simulink model "Australian14gen_original"  (R2017a)
settings: Solver=ode23tb  StartTime=0.0  StopTime=70  MaxStep=1/60  RelTol=1e-3  AbsTol=1e-1  EnableMultiTasking=on
PreLoadFcn:
  | dataaustralian14gen
values from neighbouring files (symbols this model uses):
  bus_v = [ 101	15 ... (first row only)    [dataaustralian14gen.m]
  comp = [ 1	211	0	0 ... (first row only)    [dataaustralian14gen.m]
  Exc = [ 101	0	 200	0.1	    13.25  2.5	 0	0       0       0       0       0 ... (first row only)    [dataaustralian14gen.m]
  FH = 13    [dataaustralian14gen.m]
  FI = 1    [dataaustralian14gen.m]
  FL = .1    (= 0.1)    [dataaustralian14gen.m]
  G_data = [ 101	333.3	15	3.6	0.14	1.1	0.65	0.25	8.5     0.25	0.05	0       0       0.25	0.2 	0 ... (first row only)    [dataaustralian14gen.m]
  KH = 120    [dataaustralian14gen.m]
  KI = 10    [dataaustralian14gen.m]
  KL = 10    [dataaustralian14gen.m]
  line = [ 102	217	0.0084	0.0667	0.817	330	1 ... (first row only)    [dataaustralian14gen.m]
  p = p_case4    [dataaustralian14gen.m]
  PSSMODEL = 1    [dataaustralian14gen.m]
  trans = [ 1	101	102	15	330	333.3	12	12 ... (first row only)    [dataaustralian14gen.m]
undefined symbols (not defined in the file or in its folder): D1, Delta
libraries: powerlib x297, sps_avr x14, factslib x5, powerlib_extras x4
(part 1 of 3)
Description:
  | SimPowerSystem model of the Simplified 14-Generator model
  | of the SE Australian Power System developed by Mike Gibbard & David Vowles,
  | School of Electrical & Electronic Engineering, The university of Adelaide, south australia)
  | 
  | SimPowerSystems model and validations by Ali Moeini and Innocent Kamwa,
  | IREQ, Hydro-Québec, Canada
settings Model: Creator=IREQ  LastModifiedBy=dominic
settings DataIOCC: LimitDataPoints=on  SaveFormat=Array
settings OptimizationCC: ExpressionDepthLimit=2147483647  LifeSpan=inf
settings DebuggingCC: UnderspecifiedInitializationDetection=Classic  MergeDetectMultiDrivingBlocksExec=none  IgnoredZcDiagnostic=none  SolverPrmCheckMsg=warning  UnconnectedInputMsg=none  UnconnectedOutputMsg=none  UnconnectedLineMsg=none  StateNameClashWarn=warning  SFUnexpectedBacktrackingDiag=warning  SFNoUnconditionalDefaultTransitionDiag=warning  SFExecutionAtInitializationDiag=none
settings HardwareCC: ProdBitPerPointer=32  ProdBitPerSizeT=32  ProdBitPerPtrDiffT=32  ProdLargestAtomicFloat=None  ProdIntDivRoundTo=Undefined  ProdEndianess=Unspecified  ProdWordSize=32  ProdHWDeviceType=32-bit Generic
settings ModelReferenceCC: PropagateSignalLabelsOutOfModel=off
settings GRTTargetCC: TargetLangStandard=C89/C90 (ANSI)  GeneratePreprocessorConditionals=Disable all
settings ConfigComp: CovMetricSettings=dw  CovHtmlReporting=on  CovSaveCumulativeToWorkspaceVar=on  CovSaveSingleToWorkspaceVar=on  CovExternalEMLEnable=off  CovSFcnEnable=off

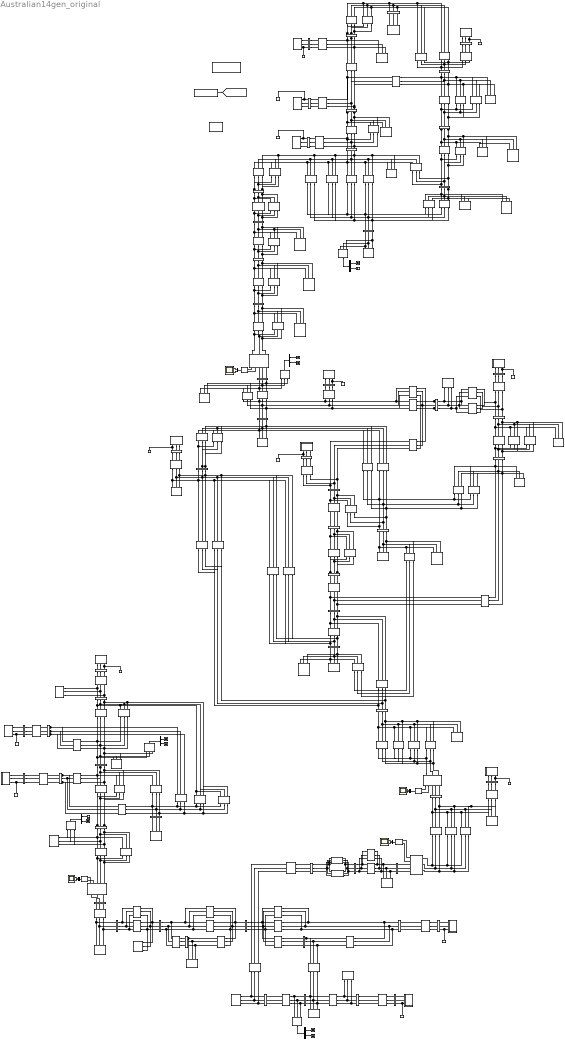
== system Australian14gen_original ==
  1 : powerlib/Elements/Three-Phase Series RLC Branch  LConnTagsString=A|B|C  RConnTagsString=A|B|C  BranchType=C  Resistance=0  Inductance=0  Capacitance=1/(0.0337)/(2*pi*50)*(330^2/100)  Measurements=None
  2 : powerlib/Elements/Three-Phase Series RLC Branch  LConnTagsString=A|B|C  RConnTagsString=A|B|C  BranchType=C  Resistance=0  Inductance=0  Capacitance=1/(0.0337)/(2*pi*50)*(330^2/100)  Measurements=None
  3-Phase Active & Reactive Power (Phasor Type){1..4} (4 alike) : powerlib_extras/Phasor Library/3-Phase Active & Reactive Power (Phasor Type)
      settings: SourceProductName=The database /home/dominic/.matlab/R2017a/slblocks_master.db is locked, or a table in the database is locked. (database is locked)
  B101 : powerlib/Measurements/Three-Phase V-I Measurement  VoltageMeasurement=phase-to-phase  SetLabelV=on  LabelV=Vabc_B101  Vpu=off  VpuLL=off  CurrentMeasurement=no  SetLabelI=on  LabelI=Iabc_B101  Ipu=off  Pbase=100e6  Vbase=bus_v(1,2)*e3  OutputType=Complex  PhasorSimulation=on  PSBequivalent=0
  B102 : powerlib/Measurements/Three-Phase V-I Measurement  VoltageMeasurement=phase-to-ground  SetLabelV=on  LabelV=Vabc_B102  Vpu=off  VpuLL=off  CurrentMeasurement=yes  SetLabelI=on  LabelI=Iabc_B102  Ipu=off  Pbase=100e6  Vbase=bus_v(2,2)*e3  OutputType=Complex  PhasorSimulation=on  PSBequivalent=0
  B201 : powerlib/Measurements/Three-Phase V-I Measurement  VoltageMeasurement=phase-to-phase  SetLabelV=on  LabelV=Vabc_B201  Vpu=off  VpuLL=off  CurrentMeasurement=no  SetLabelI=on  LabelI=Iabc_B201  Ipu=off  Pbase=100e6  Vbase=bus_v(3,2)*e3  OutputType=Complex  PhasorSimulation=on  PSBequivalent=0
  B202 : powerlib/Measurements/Three-Phase V-I Measurement  VoltageMeasurement=phase-to-phase  SetLabelV=on  LabelV=Vabc_B202  Vpu=off  VpuLL=off  CurrentMeasurement=no  SetLabelI=on  LabelI=Iabc_B202  Ipu=off  Pbase=100e6  Vbase=bus_v(4,2)*e3  OutputType=Complex  PhasorSimulation=on  PSBequivalent=0
  B203 : powerlib/Measurements/Three-Phase V-I Measurement  VoltageMeasurement=phase-to-phase  SetLabelV=on  LabelV=Vabc_B203  Vpu=off  VpuLL=off  CurrentMeasurement=no  SetLabelI=on  LabelI=Iabc_B203  Ipu=off  Pbase=100e6  Vbase=bus_v(5,2)*e3  OutputType=Complex  PhasorSimulation=on  PSBequivalent=0
  B204 : powerlib/Measurements/Three-Phase V-I Measurement  VoltageMeasurement=phase-to-phase  SetLabelV=on  LabelV=Vabc_B204  Vpu=off  VpuLL=off  CurrentMeasurement=no  SetLabelI=on  LabelI=Iabc_B204  Ipu=off  Pbase=100e6  Vbase=bus_v(6,2)*e3  OutputType=Complex  PhasorSimulation=on  PSBequivalent=0
  B205 : powerlib/Measurements/Three-Phase V-I Measurement  VoltageMeasurement=phase-to-ground  SetLabelV=on  LabelV=Vabc_B205  Vpu=off  VpuLL=off  CurrentMeasurement=yes  SetLabelI=on  LabelI=Iabc_B205  Ipu=off  Pbase=100e6  Vbase=bus_v(7,2)*e3  OutputType=Complex  PhasorSimulation=on  PSBequivalent=0
  B206 : powerlib/Measurements/Three-Phase V-I Measurement  VoltageMeasurement=phase-to-ground  SetLabelV=on  LabelV=Vabc_B206  Vpu=off  VpuLL=off  CurrentMeasurement=yes  SetLabelI=on  LabelI=Iabc_B206  Ipu=off  Pbase=100e6  Vbase=bus_v(8,2)*e3  OutputType=Complex  PhasorSimulation=on  PSBequivalent=0
  B207 : powerlib/Measurements/Three-Phase V-I Measurement  VoltageMeasurement=phase-to-ground  SetLabelV=on  LabelV=Vabc_B207  Vpu=off  VpuLL=off  CurrentMeasurement=yes  SetLabelI=on  LabelI=Iabc_B207  Ipu=off  Pbase=100e6  Vbase=138e3  OutputType=Complex  PhasorSimulation=on  PSBequivalent=0
  B208 : powerlib/Measurements/Three-Phase V-I Measurement  VoltageMeasurement=phase-to-ground  SetLabelV=on  LabelV=Vabc_B208  Vpu=off  VpuLL=off  CurrentMeasurement=yes  SetLabelI=on  LabelI=Iabc_B208  Ipu=off  Pbase=100e6  Vbase=138e3  OutputType=Complex  PhasorSimulation=on  PSBequivalent=0
  B209 : powerlib/Measurements/Three-Phase V-I Measurement  VoltageMeasurement=phase-to-ground  SetLabelV=on  LabelV=Vabc_B209  Vpu=off  VpuLL=off  CurrentMeasurement=yes  SetLabelI=on  LabelI=Iabc_B209  Ipu=off  Pbase=100e6  Vbase=138e3  OutputType=Complex  PhasorSimulation=on  PSBequivalent=0
  B210 : powerlib/Measurements/Three-Phase V-I Measurement  VoltageMeasurement=phase-to-ground  SetLabelV=on  LabelV=Vabc_B210  Vpu=off  VpuLL=off  CurrentMeasurement=yes  SetLabelI=on  LabelI=Iabc_B210  Ipu=off  Pbase=100e6  Vbase=138e3  OutputType=Complex  PhasorSimulation=on  PSBequivalent=0
  B211 : powerlib/Measurements/Three-Phase V-I Measurement  VoltageMeasurement=phase-to-ground  SetLabelV=on  LabelV=Vabc_B211  Vpu=off  VpuLL=off  CurrentMeasurement=yes  SetLabelI=on  LabelI=Iabc_B211  Ipu=off  Pbase=100e6  Vbase=138e3  OutputType=Complex  PhasorSimulation=on  PSBequivalent=0
  B212 : powerlib/Measurements/Three-Phase V-I Measurement  VoltageMeasurement=phase-to-ground  SetLabelV=on  LabelV=Vabc_B212  Vpu=off  VpuLL=off  CurrentMeasurement=yes  SetLabelI=on  LabelI=Iabc_B212  Ipu=off  Pbase=100e6  Vbase=138e3  OutputType=Complex  PhasorSimulation=on  PSBequivalent=0
  B213 : powerlib/Measurements/Three-Phase V-I Measurement  VoltageMeasurement=phase-to-ground  SetLabelV=on  LabelV=Vabc_B213  Vpu=off  VpuLL=off  CurrentMeasurement=yes  SetLabelI=on  LabelI=Iabc_B213  Ipu=off  Pbase=100e6  Vbase=138e3  OutputType=Complex  PhasorSimulation=on  PSBequivalent=0
  B214 : powerlib/Measurements/Three-Phase V-I Measurement  VoltageMeasurement=phase-to-ground  SetLabelV=on  LabelV=Vabc_B214  Vpu=off  VpuLL=off  CurrentMeasurement=yes  SetLabelI=on  LabelI=Iabc_B214  Ipu=off  Pbase=100e6  Vbase=138e3  OutputType=Complex  PhasorSimulation=on  PSBequivalent=0
  B215 : powerlib/Measurements/Three-Phase V-I Measurement  VoltageMeasurement=phase-to-ground  SetLabelV=on  LabelV=Vabc_B215  Vpu=off  VpuLL=off  CurrentMeasurement=yes  SetLabelI=on  LabelI=Iabc_B215  Ipu=off  Pbase=100e6  Vbase=138e3  OutputType=Complex  PhasorSimulation=on  PSBequivalent=0
  B216 : powerlib/Measurements/Three-Phase V-I Measurement  VoltageMeasurement=phase-to-ground  SetLabelV=on  LabelV=Vabc_B216  Vpu=off  VpuLL=off  CurrentMeasurement=yes  SetLabelI=on  LabelI=Iabc_B216  Ipu=off  Pbase=100e6  Vbase=138e3  OutputType=Complex  PhasorSimulation=on  PSBequivalent=0
  B217 : powerlib/Measurements/Three-Phase V-I Measurement  VoltageMeasurement=phase-to-ground  SetLabelV=on  LabelV=Vabc_B217  Vpu=off  VpuLL=off  CurrentMeasurement=yes  SetLabelI=on  LabelI=Iabc_B217  Ipu=off  Pbase=100e6  Vbase=138e3  OutputType=Complex  PhasorSimulation=on  PSBequivalent=0
  B301 : powerlib/Measurements/Three-Phase V-I Measurement  VoltageMeasurement=phase-to-phase  SetLabelV=on  LabelV=Vabc_B301  Vpu=off  VpuLL=off  CurrentMeasurement=no  SetLabelI=on  LabelI=Iabc_B301  Ipu=off  Pbase=100e6  Vbase=138e3  OutputType=Complex  PhasorSimulation=on  PSBequivalent=0
  B302 : powerlib/Measurements/Three-Phase V-I Measurement  VoltageMeasurement=phase-to-phase  SetLabelV=on  LabelV=Vabc_B302  Vpu=off  VpuLL=off  CurrentMeasurement=no  SetLabelI=on  LabelI=Iabc_B302  Ipu=off  Pbase=100e6  Vbase=138e3  OutputType=Complex  PhasorSimulation=on  PSBequivalent=0
  B303 : powerlib/Measurements/Three-Phase V-I Measurement  VoltageMeasurement=phase-to-ground  SetLabelV=on  LabelV=Vabc_B303  Vpu=off  VpuLL=off  CurrentMeasurement=yes  SetLabelI=on  LabelI=Iabc_B303  Ipu=off  Pbase=100e6  Vbase=138e3  OutputType=Complex  PhasorSimulation=on  PSBequivalent=0
  B304 : powerlib/Measurements/Three-Phase V-I Measurement  VoltageMeasurement=phase-to-ground  SetLabelV=on  LabelV=Vabc_B304  Vpu=off  VpuLL=off  CurrentMeasurement=yes  SetLabelI=on  LabelI=Iabc_B304  Ipu=off  Pbase=100e6  Vbase=138e3  OutputType=Complex  PhasorSimulation=on  PSBequivalent=0
  B305 : powerlib/Measurements/Three-Phase V-I Measurement  VoltageMeasurement=phase-to-ground  SetLabelV=on  LabelV=Vabc_B305  Vpu=off  VpuLL=off  CurrentMeasurement=yes  SetLabelI=on  LabelI=Iabc_B305  Ipu=off  Pbase=100e6  Vbase=138e3  OutputType=Complex  PhasorSimulation=on  PSBequivalent=0
  B306 : powerlib/Measurements/Three-Phase V-I Measurement  VoltageMeasurement=phase-to-ground  SetLabelV=on  LabelV=Vabc_B306  Vpu=off  VpuLL=off  CurrentMeasurement=yes  SetLabelI=on  LabelI=Iabc_B306  Ipu=off  Pbase=100e6  Vbase=138e3  OutputType=Complex  PhasorSimulation=on  PSBequivalent=0
  B307 : powerlib/Measurements/Three-Phase V-I Measurement  VoltageMeasurement=phase-to-ground  SetLabelV=on  LabelV=Vabc_B307  Vpu=off  VpuLL=off  CurrentMeasurement=yes  SetLabelI=on  LabelI=Iabc_B307  Ipu=off  Pbase=100e6  Vbase=138e3  OutputType=Complex  PhasorSimulation=on  PSBequivalent=0
  B308 : powerlib/Measurements/Three-Phase V-I Measurement  VoltageMeasurement=phase-to-ground  SetLabelV=on  LabelV=Vabc_B308  Vpu=off  VpuLL=off  CurrentMeasurement=yes  SetLabelI=on  LabelI=Iabc_B308  Ipu=off  Pbase=100e6  Vbase=138e3  OutputType=Complex  PhasorSimulation=on  PSBequivalent=0
  B309 : powerlib/Measurements/Three-Phase V-I Measurement  VoltageMeasurement=phase-to-ground  SetLabelV=on  LabelV=Vabc_B309  Vpu=off  VpuLL=off  CurrentMeasurement=yes  SetLabelI=on  LabelI=Iabc_B309  Ipu=off  Pbase=100e6  Vbase=138e3  OutputType=Complex  PhasorSimulation=on  PSBequivalent=0
  B310 : powerlib/Measurements/Three-Phase V-I Measurement  VoltageMeasurement=phase-to-ground  SetLabelV=on  LabelV=Vabc_B310  Vpu=off  VpuLL=off  CurrentMeasurement=yes  SetLabelI=on  LabelI=Iabc_B310  Ipu=off  Pbase=100e6  Vbase=138e3  OutputType=Complex  PhasorSimulation=on  PSBequivalent=0
  B311 : powerlib/Measurements/Three-Phase V-I Measurement  VoltageMeasurement=phase-to-ground  SetLabelV=on  LabelV=Vabc_B311  Vpu=off  VpuLL=off  CurrentMeasurement=yes  SetLabelI=on  LabelI=Iabc_B311  Ipu=off  Pbase=100e6  Vbase=138e3  OutputType=Complex  PhasorSimulation=on  PSBequivalent=0
  B312 : powerlib/Measurements/Three-Phase V-I Measurement  VoltageMeasurement=phase-to-ground  SetLabelV=on  LabelV=Vabc_B312  Vpu=off  VpuLL=off  CurrentMeasurement=yes  SetLabelI=on  LabelI=Iabc_B312  Ipu=off  Pbase=100e6  Vbase=138e3  OutputType=Complex  PhasorSimulation=on  PSBequivalent=0
  B313 : powerlib/Measurements/Three-Phase V-I Measurement  VoltageMeasurement=phase-to-ground  SetLabelV=on  LabelV=Vabc_B313  Vpu=off  VpuLL=off  CurrentMeasurement=yes  SetLabelI=on  LabelI=Iabc_B313  Ipu=off  Pbase=100e6  Vbase=138e3  OutputType=Complex  PhasorSimulation=on  PSBequivalent=0
  B314 : powerlib/Measurements/Three-Phase V-I Measurement  VoltageMeasurement=phase-to-ground  SetLabelV=on  LabelV=Vabc_B314  Vpu=off  VpuLL=off  CurrentMeasurement=yes  SetLabelI=on  LabelI=Iabc_B314  Ipu=off  Pbase=100e6  Vbase=138e3  OutputType=Complex  PhasorSimulation=on  PSBequivalent=0
  B315 : powerlib/Measurements/Three-Phase V-I Measurement  VoltageMeasurement=phase-to-ground  SetLabelV=on  LabelV=Vabc_B315  Vpu=off  VpuLL=off  CurrentMeasurement=yes  SetLabelI=on  LabelI=Iabc_B315  Ipu=off  Pbase=100e6  Vbase=138e3  OutputType=Complex  PhasorSimulation=on  PSBequivalent=0
  B401 : powerlib/Measurements/Three-Phase V-I Measurement  VoltageMeasurement=phase-to-phase  SetLabelV=on  LabelV=Vabc_B401  Vpu=off  VpuLL=off  CurrentMeasurement=no  SetLabelI=on  LabelI=Iabc_B401  Ipu=off  Pbase=100e6  Vbase=138e3  OutputType=Complex  PhasorSimulation=on  PSBequivalent=0
  B402 : powerlib/Measurements/Three-Phase V-I Measurement  VoltageMeasurement=phase-to-phase  SetLabelV=on  LabelV=Vabc_B402  Vpu=off  VpuLL=off  CurrentMeasurement=no  SetLabelI=on  LabelI=Iabc_B402  Ipu=off  Pbase=100e6  Vbase=138e3  OutputType=Complex  PhasorSimulation=on  PSBequivalent=0
  B403 : powerlib/Measurements/Three-Phase V-I Measurement  VoltageMeasurement=phase-to-phase  SetLabelV=on  LabelV=Vabc_B403  Vpu=off  VpuLL=off  CurrentMeasurement=no  SetLabelI=on  LabelI=Iabc_B403  Ipu=off  Pbase=100e6  Vbase=138e3  OutputType=Complex  PhasorSimulation=on  PSBequivalent=0
  B404 : powerlib/Measurements/Three-Phase V-I Measurement  VoltageMeasurement=phase-to-phase  SetLabelV=on  LabelV=Vabc_B404  Vpu=off  VpuLL=off  CurrentMeasurement=no  SetLabelI=on  LabelI=Iabc_B404  Ipu=off  Pbase=100e6  Vbase=138e3  OutputType=Complex  PhasorSimulation=on  PSBequivalent=0
  B405 : powerlib/Measurements/Three-Phase V-I Measurement  VoltageMeasurement=phase-to-ground  SetLabelV=on  LabelV=Vabc_B405  Vpu=off  VpuLL=off  CurrentMeasurement=yes  SetLabelI=on  LabelI=Iabc_B405  Ipu=off  Pbase=100e6  Vbase=138e3  OutputType=Complex  PhasorSimulation=on  PSBequivalent=0
  B406 : powerlib/Measurements/Three-Phase V-I Measurement  VoltageMeasurement=phase-to-ground  SetLabelV=on  LabelV=Vabc_B406  Vpu=off  VpuLL=off  CurrentMeasurement=yes  SetLabelI=on  LabelI=Iabc_B406  Ipu=off  Pbase=100e6  Vbase=138e3  OutputType=Complex  PhasorSimulation=on  PSBequivalent=0
  B407 : powerlib/Measurements/Three-Phase V-I Measurement  VoltageMeasurement=phase-to-ground  SetLabelV=on  LabelV=Vabc_B407  Vpu=off  VpuLL=off  CurrentMeasurement=yes  SetLabelI=on  LabelI=Iabc_B407  Ipu=off  Pbase=100e6  Vbase=138e3  OutputType=Complex  PhasorSimulation=on  PSBequivalent=0
  B408 : powerlib/Measurements/Three-Phase V-I Measurement  VoltageMeasurement=phase-to-ground  SetLabelV=on  LabelV=Vabc_B408  Vpu=off  VpuLL=off  CurrentMeasurement=yes  SetLabelI=on  LabelI=Iabc_B408  Ipu=off  Pbase=100e6  Vbase=138e3  OutputType=Complex  PhasorSimulation=on  PSBequivalent=0
  B409 : powerlib/Measurements/Three-Phase V-I Measurement  VoltageMeasurement=phase-to-ground  SetLabelV=on  LabelV=Vabc_B409  Vpu=off  VpuLL=off  CurrentMeasurement=yes  SetLabelI=on  LabelI=Iabc_B409  Ipu=off  Pbase=100e6  Vbase=138e3  OutputType=Complex  PhasorSimulation=on  PSBequivalent=0
  B410 : powerlib/Measurements/Three-Phase V-I Measurement  VoltageMeasurement=phase-to-ground  SetLabelV=on  LabelV=Vabc_B410  Vpu=off  VpuLL=off  CurrentMeasurement=yes  SetLabelI=on  LabelI=Iabc_B410  Ipu=off  Pbase=100e6  Vbase=138e3  OutputType=Complex  PhasorSimulation=on  PSBequivalent=0
  B411 : powerlib/Measurements/Three-Phase V-I Measurement  VoltageMeasurement=phase-to-ground  SetLabelV=on  LabelV=Vabc_B411  Vpu=off  VpuLL=off  CurrentMeasurement=yes  SetLabelI=on  LabelI=Iabc_B411  Ipu=off  Pbase=100e6  Vbase=138e3  OutputType=Complex  PhasorSimulation=on  PSBequivalent=0
  B412 : powerlib/Measurements/Three-Phase V-I Measurement  VoltageMeasurement=phase-to-ground  SetLabelV=on  LabelV=Vabc_B412  Vpu=off  VpuLL=off  CurrentMeasurement=yes  SetLabelI=on  LabelI=Iabc_B412  Ipu=off  Pbase=100e6  Vbase=138e3  OutputType=Complex  PhasorSimulation=on  PSBequivalent=0
  B413 : powerlib/Measurements/Three-Phase V-I Measurement  VoltageMeasurement=phase-to-ground  SetLabelV=on  LabelV=Vabc_B413  Vpu=off  VpuLL=off  CurrentMeasurement=yes  SetLabelI=on  LabelI=Iabc_B413  Ipu=off  Pbase=100e6  Vbase=138e3  OutputType=Complex  PhasorSimulation=on  PSBequivalent=0
  B414 : powerlib/Measurements/Three-Phase V-I Measurement  VoltageMeasurement=phase-to-ground  SetLabelV=on  LabelV=Vabc_B414  Vpu=off  VpuLL=off  CurrentMeasurement=yes  SetLabelI=on  LabelI=Iabc_B414  Ipu=off  Pbase=100e6  Vbase=138e3  OutputType=Complex  PhasorSimulation=on  PSBequivalent=0
  B415 : powerlib/Measurements/Three-Phase V-I Measurement  VoltageMeasurement=phase-to-ground  SetLabelV=on  LabelV=Vabc_B415  Vpu=off  VpuLL=off  CurrentMeasurement=yes  SetLabelI=on  LabelI=Iabc_B415  Ipu=off  Pbase=100e6  Vbase=138e3  OutputType=Complex  PhasorSimulation=on  PSBequivalent=0
  B416 : powerlib/Measurements/Three-Phase V-I Measurement  VoltageMeasurement=phase-to-ground  SetLabelV=on  LabelV=Vabc_B416  Vpu=off  VpuLL=off  CurrentMeasurement=yes  SetLabelI=on  LabelI=Iabc_B416  Ipu=off  Pbase=100e6  Vbase=138e3  OutputType=Complex  PhasorSimulation=on  PSBequivalent=0
  B501 : powerlib/Measurements/Three-Phase V-I Measurement  VoltageMeasurement=phase-to-phase  SetLabelV=on  LabelV=Vabc_B501  Vpu=off  VpuLL=off  CurrentMeasurement=no  SetLabelI=on  LabelI=Iabc_B501  Ipu=off  Pbase=100e6  Vbase=138e3  OutputType=Complex  PhasorSimulation=on  PSBequivalent=0
  B502 : powerlib/Measurements/Three-Phase V-I Measurement  VoltageMeasurement=no  SetLabelV=on  LabelV=Vabc_B502  Vpu=off  VpuLL=off  CurrentMeasurement=no  SetLabelI=on  LabelI=Iabc_B502  Ipu=off  Pbase=100e6  Vbase=138e3  OutputType=Complex  PhasorSimulation=on  PSBequivalent=0
  B503 : powerlib/Measurements/Three-Phase V-I Measurement  VoltageMeasurement=phase-to-phase  SetLabelV=on  LabelV=Vabc_B503  Vpu=off  VpuLL=off  CurrentMeasurement=yes  SetLabelI=on  LabelI=Iabc_B503  Ipu=off  Pbase=100e6  Vbase=138e3  OutputType=Complex  PhasorSimulation=on  PSBequivalent=0
  B504 : powerlib/Measurements/Three-Phase V-I Measurement  VoltageMeasurement=phase-to-ground  SetLabelV=on  LabelV=Vabc_B504  Vpu=off  VpuLL=off  CurrentMeasurement=yes  SetLabelI=on  LabelI=Iabc_B504  Ipu=off  Pbase=100e6  Vbase=138e3  OutputType=Complex  PhasorSimulation=on  PSBequivalent=0
  B505 : powerlib/Measurements/Three-Phase V-I Measurement  VoltageMeasurement=phase-to-ground  SetLabelV=on  LabelV=Vabc_B505  Vpu=off  VpuLL=off  CurrentMeasurement=yes  SetLabelI=on  LabelI=Iabc_B505  Ipu=off  Pbase=100e6  Vbase=138e3  OutputType=Complex  PhasorSimulation=on  PSBequivalent=0
  B506 : powerlib/Measurements/Three-Phase V-I Measurement  VoltageMeasurement=phase-to-ground  SetLabelV=on  LabelV=Vabc_B506  Vpu=off  VpuLL=off  CurrentMeasurement=yes  SetLabelI=on  LabelI=Iabc_B506  Ipu=off  Pbase=100e6  Vbase=138e3  OutputType=Complex  PhasorSimulation=on  PSBequivalent=0
  B507 : powerlib/Measurements/Three-Phase V-I Measurement  VoltageMeasurement=phase-to-ground  SetLabelV=on  LabelV=Vabc_B507  Vpu=off  VpuLL=off  CurrentMeasurement=yes  SetLabelI=on  LabelI=Iabc_B507  Ipu=off  Pbase=100e6  Vbase=138e3  OutputType=Complex  PhasorSimulation=on  PSBequivalent=0
  B508 : powerlib/Measurements/Three-Phase V-I Measurement  VoltageMeasurement=phase-to-ground  SetLabelV=on  LabelV=Vabc_B508  Vpu=off  VpuLL=off  CurrentMeasurement=yes  SetLabelI=on  LabelI=Iabc_B508  Ipu=off  Pbase=100e6  Vbase=138e3  OutputType=Complex  PhasorSimulation=on  PSBequivalent=0
  B509 : powerlib/Measurements/Three-Phase V-I Measurement  VoltageMeasurement=phase-to-ground  SetLabelV=on  LabelV=Vabc_B3509  Vpu=off  VpuLL=off  CurrentMeasurement=yes  SetLabelI=on  LabelI=Iabc_B509  Ipu=off  Pbase=100e6  Vbase=138e3  OutputType=Complex  PhasorSimulation=on  PSBequivalent=0
  BPS_2 : Subsystem
  Bus Selector{1..5} (5 alike) : BusSelector  OutputSignals=Control.Q (pu),Control.Vm (pu)
  CPS_4 : Subsystem
  Comp2-212 : powerlib/Elements/Three-Phase Parallel RLC Load  LConnTagsString=A|B|C  Configuration=Y (grounded)  NominalVoltage=(330000)*1  Vabc=[1e3 1e3 1e3]  Vabcp=[1e3 1e3 1e3]  NominalFrequency=50  UnbalancedPower=off  ActivePower=0  InductivePower=comp(2,3)*1e6  CapacitivePower=comp(2,4)*1e6  Pabc=[10e3 9e3 11e3]  QLabc=[100 90 110]  QCabc=[100 90 110]  Pabcp=[10e3 9e3 11e3]  QLabcp=[100 90 110]  QCabcp=[100 90 110]  Measurements=None  LoadType=constant Z
  Comp3-216 : powerlib/Elements/Three-Phase Parallel RLC Load  LConnTagsString=A|B|C  Configuration=Y (grounded)  NominalVoltage=(330000)*1  Vabc=[1e3 1e3 1e3]  Vabcp=[1e3 1e3 1e3]  NominalFrequency=50  UnbalancedPower=off  ActivePower=0  InductivePower=comp(3,3)*1e6  CapacitivePower=comp(3,4)*1e6  Pabc=[10e3 9e3 11e3]  QLabc=[100 90 110]  QCabc=[100 90 110]  Pabcp=[10e3 9e3 11e3]  QLabcp=[100 90 110]  QCabcp=[100 90 110]  Measurements=None  LoadType=constant Z
  Comp4-409 : powerlib/Elements/Three-Phase Parallel RLC Load  LConnTagsString=A|B|C  Configuration=Y (grounded)  NominalVoltage=(275000)*1  Vabc=[1e3 1e3 1e3]  Vabcp=[1e3 1e3 1e3]  NominalFrequency=50  UnbalancedPower=off  ActivePower=0  InductivePower=comp(4,3)*1e6  CapacitivePower=comp(4,4)*1e6  Pabc=[10e3 9e3 11e3]  QLabc=[100 90 110]  QCabc=[100 90 110]  Pabcp=[10e3 9e3 11e3]  QLabcp=[100 90 110]  QCabcp=[100 90 110]  Measurements=None  LoadType=constant Z
  Comp5-411 : powerlib/Elements/Three-Phase Parallel RLC Load  LConnTagsString=A|B|C  Configuration=Y (grounded)  NominalVoltage=(275000)*1  Vabc=[1e3 1e3 1e3]  Vabcp=[1e3 1e3 1e3]  NominalFrequency=50  UnbalancedPower=off  ActivePower=0  InductivePower=comp(5,3)*1e6  CapacitivePower=comp(5,4)*1e6  Pabc=[10e3 9e3 11e3]  QLabc=[100 90 110]  QCabc=[100 90 110]  Pabcp=[10e3 9e3 11e3]  QLabcp=[100 90 110]  QCabcp=[100 90 110]  Measurements=None  LoadType=constant Z
  Comp6-414 : powerlib/Elements/Three-Phase Parallel RLC Load  LConnTagsString=A|B|C  Configuration=Y (grounded)  NominalVoltage=(330000)*1  Vabc=[1e3 1e3 1e3]  Vabcp=[1e3 1e3 1e3]  NominalFrequency=50  UnbalancedPower=off  ActivePower=0  InductivePower=comp(6,3)*1e6  CapacitivePower=comp(6,4)*1e6  Pabc=[10e3 9e3 11e3]  QLabc=[100 90 110]  QCabc=[100 90 110]  Pabcp=[10e3 9e3 11e3]  QLabcp=[100 90 110]  QCabcp=[100 90 110]  Measurements=None  LoadType=constant Z
  Comp7-415 : powerlib/Elements/Three-Phase Parallel RLC Load  LConnTagsString=A|B|C  Configuration=Y (grounded)  NominalVoltage=(330000)*1  Vabc=[1e3 1e3 1e3]  Vabcp=[1e3 1e3 1e3]  NominalFrequency=50  UnbalancedPower=off  ActivePower=0  InductivePower=comp(7,3)*1e6  CapacitivePower=comp(7,4)*1e6  Pabc=[10e3 9e3 11e3]  QLabc=[100 90 110]  QCabc=[100 90 110]  Pabcp=[10e3 9e3 11e3]  QLabcp=[100 90 110]  QCabcp=[100 90 110]  Measurements=None  LoadType=constant Z
  Comp8-416 : powerlib/Elements/Three-Phase Parallel RLC Load  LConnTagsString=A|B|C  Configuration=Y (grounded)  NominalVoltage=(330000)*1  Vabc=[1e3 1e3 1e3]  Vabcp=[1e3 1e3 1e3]  NominalFrequency=50  UnbalancedPower=off  ActivePower=0  InductivePower=comp(8,3)*1e6  CapacitivePower=comp(8,4)*1e6  Pabc=[10e3 9e3 11e3]  QLabc=[100 90 110]  QCabc=[100 90 110]  Pabcp=[10e3 9e3 11e3]  QLabcp=[100 90 110]  QCabcp=[100 90 110]  Measurements=None  LoadType=constant Z
  Demux{,1..3} (4 alike) : Demux  Outputs=2
  EPS_2 : Subsystem
  GPS_4 : Subsystem
  HPS_1 : Subsystem
  L-1-1 : powerlib/Elements/Three-Phase PI Section Line  LConnTagsString=a|b|c  RConnTagsString=A|B|C  Frequency=50  Resistances="[ line(1,3)  line(1,3)*3]"  Inductances="[ line(1,4)  line(1,4)*3]"  Capacitances="[ line(1,5)  line(1,5)/3]"  Length=1
      settings: SourceProductName=Simscape Power Systems
  L-1-2 : powerlib/Elements/Three-Phase PI Section Line  LConnTagsString=a|b|c  RConnTagsString=A|B|C  Frequency=50  Resistances="[ line(1,3)  line(1,3)*3]"  Inductances="[ line(1,4)  line(1,4)*3]"  Capacitances="[ line(1,5)  line(1,5)/3]"  Length=1
      settings: SourceProductName=Simscape Power Systems
  L-10-1 : powerlib/Elements/Three-Phase PI Section Line  LConnTagsString=a|b|c  RConnTagsString=A|B|C  Frequency=50  Resistances="[ line(10,3)  line(10,3)*3]"  Inductances="[ line(10,4)  line(10,4)*3]"  Capacitances="[ line(10,5)  line(10,5)/3]"  Length=1
      settings: SourceProductName=Simscape Power Systems
  L-10-2 : powerlib/Elements/Three-Phase PI Section Line  LConnTagsString=a|b|c  RConnTagsString=A|B|C  Frequency=50  Resistances="[ line(10,3)  line(10,3)*3]"  Inductances="[ line(10,4)  line(10,4)*3]"  Capacitances="[ line(10,5)  line(10,5)/3]"  Length=1
      settings: SourceProductName=Simscape Power Systems
  L-11 : powerlib/Elements/Three-Phase PI Section Line  LConnTagsString=a|b|c  RConnTagsString=A|B|C  Frequency=50  Resistances="[ line(11,3)  line(11,3)*3]"  Inductances="[ line(11,4)  line(11,4)*3]"  Capacitances="[ line(11,5)  line(11,5)/3]"  Length=1
      settings: SourceProductName=Simscape Power Systems
  L-12-1 : powerlib/Elements/Three-Phase PI Section Line  LConnTagsString=a|b|c  RConnTagsString=A|B|C  Frequency=50  Resistances="[ line(12,3)  line(12,3)*3]"  Inductances="[ line(12,4)  line(12,4)*3]"  Capacitances="[ line(12,5)  line(12,5)/3]"  Length=1
      settings: SourceProductName=Simscape Power Systems
  L-12-2 : powerlib/Elements/Three-Phase PI Section Line  LConnTagsString=a|b|c  RConnTagsString=A|B|C  Frequency=50  Resistances="[ line(12,3)  line(12,3)*3]"  Inductances="[ line(12,4)  line(12,4)*3]"  Capacitances="[ line(12,5)  line(12,5)/3]"  Length=1
      settings: SourceProductName=Simscape Power Systems
  L-12-3 : powerlib/Elements/Three-Phase PI Section Line  LConnTagsString=a|b|c  RConnTagsString=A|B|C  Frequency=50  Resistances="[ line(12,3)  line(12,3)*3]"  Inductances="[ line(12,4)  line(12,4)*3]"  Capacitances="[ line(12,5)  line(12,5)/3]"  Length=1
      settings: SourceProductName=Simscape Power Systems
  L-13 : powerlib/Elements/Three-Phase PI Section Line  LConnTagsString=a|b|c  RConnTagsString=A|B|C  Frequency=50  Resistances="[ line(13,3)  line(13,3)*3]"  Inductances="[ line(13,4)  line(13,4)*3]"  Capacitances="[ line(13,5)  line(13,5)/3]"  Length=1
      settings: SourceProductName=Simscape Power Systems
  L-14-1 : powerlib/Elements/Three-Phase PI Section Line  LConnTagsString=a|b|c  RConnTagsString=A|B|C  Frequency=50  Resistances="[ line(14,3)  line(14,3)*3]"  Inductances="[ line(14,4)  line(14,4)*3]"  Capacitances="[ line(14,5)  line(14,5)/3]"  Length=1
      settings: SourceProductName=Simscape Power Systems
  L-14-2 : powerlib/Elements/Three-Phase PI Section Line  LConnTagsString=a|b|c  RConnTagsString=A|B|C  Frequency=50  Resistances="[ line(14,3)  line(14,3)*3]"  Inductances="[ line(14,4)  line(14,4)*3]"  Capacitances="[ line(14,5)  line(14,5)/3]"  Length=1
      settings: SourceProductName=Simscape Power Systems
  L-15-1 : powerlib/Elements/Three-Phase PI Section Line  LConnTagsString=a|b|c  RConnTagsString=A|B|C  Frequency=50  Resistances="[ line(15,3)  line(15,3)*3]"  Inductances="[ line(15,4)  line(15,4)*3]"  Capacitances="[ line(15,5)  line(15,5)/3]"  Length=1
      settings: SourceProductName=Simscape Power Systems
  L-15-2 : powerlib/Elements/Three-Phase PI Section Line  LConnTagsString=a|b|c  RConnTagsString=A|B|C  Frequency=50  Resistances="[ line(15,3)  line(15,3)*3]"  Inductances="[ line(15,4)  line(15,4)*3]"  Capacitances="[ line(15,5)  line(15,5)/3]"  Length=1
      settings: SourceProductName=Simscape Power Systems
  L-16 : powerlib/Elements/Three-Phase PI Section Line  LConnTagsString=a|b|c  RConnTagsString=A|B|C  Frequency=50  Resistances="[ line(16,3)  line(16,3)*3]"  Inductances="[ line(16,4)  line(16,4)*3]"  Capacitances="[ line(16,5)  line(16,5)/3]"  Length=1
      settings: SourceProductName=Simscape Power Systems
  L-17 : powerlib/Elements/Three-Phase PI Section Line  LConnTagsString=a|b|c  RConnTagsString=A|B|C  Frequency=50  Resistances="[ line(17,3)  line(17,3)*3]"  Inductances="[ line(17,4)  line(17,4)*3]"  Capacitances="[ line(17,5)  line(17,5)/3]"  Length=1
      settings: SourceProductName=Simscape Power Systems
  L-18 : powerlib/Elements/Three-Phase PI Section Line  LConnTagsString=a|b|c  RConnTagsString=A|B|C  Frequency=50  Resistances="[ line(18,3)  line(18,3)*3]"  Inductances="[ line(18,4)  line(18,4)*3]"  Capacitances="[ line(18,5)  line(18,5)/3]"  Length=1
      settings: SourceProductName=Simscape Power Systems
  L-19 : powerlib/Elements/Three-Phase PI Section Line  LConnTagsString=a|b|c  RConnTagsString=A|B|C  Frequency=50  Resistances="[ line(19,3)  line(19,3)*3]"  Inductances="[ line(19,4)  line(19,4)*3]"  Capacitances="[ line(19,5)  line(19,5)/3]"  Length=1
      settings: SourceProductName=Simscape Power Systems
  L-2-1 : powerlib/Elements/Three-Phase PI Section Line  LConnTagsString=a|b|c  RConnTagsString=A|B|C  Frequency=50  Resistances="[ line(2,3)  line(2,3)*3]"  Inductances="[ line(2,4)  line(2,4)*3]"  Capacitances="[ line(2,5)  line(2,5)/3]"  Length=1
      settings: SourceProductName=Simscape Power Systems
  L-2-2 : powerlib/Elements/Three-Phase PI Section Line  LConnTagsString=a|b|c  RConnTagsString=A|B|C  Frequency=50  Resistances="[ line(2,3)  line(2,3)*3]"  Inductances="[ line(2,4)  line(2,4)*3]"  Capacitances="[ line(2,5)  line(2,5)/3]"  Length=1
      settings: SourceProductName=Simscape Power Systems
  L-20-1 : powerlib/Elements/Three-Phase PI Section Line  LConnTagsString=a|b|c  RConnTagsString=A|B|C  Frequency=50  Resistances="[ line(20,3)  line(20,3)*3]"  Inductances="[ line(20,4)  line(20,4)*3]"  Capacitances="[ line(20,5)  line(20,5)/3]"  Length=1
      settings: SourceProductName=Simscape Power Systems
  L-20-2 : powerlib/Elements/Three-Phase PI Section Line  LConnTagsString=a|b|c  RConnTagsString=A|B|C  Frequency=50  Resistances="[ line(20,3)  line(20,3)*3]"  Inductances="[ line(20,4)  line(20,4)*3]"  Capacitances="[ line(20,5)  line(20,5)/3]"  Length=1
      settings: SourceProductName=Simscape Power Systems
  L-21-1 : powerlib/Elements/Three-Phase PI Section Line  LConnTagsString=a|b|c  RConnTagsString=A|B|C  Frequency=50  Resistances="[ line(21,3)  line(21,3)*3]"  Inductances="[ line(21,4)  line(21,4)*3]"  Capacitances="[ line(21,5)  line(21,5)/3]"  Length=1
      settings: SourceProductName=Simscape Power Systems
  L-21-2 : powerlib/Elements/Three-Phase PI Section Line  LConnTagsString=a|b|c  RConnTagsString=A|B|C  Frequency=50  Resistances="[ line(21,3)  line(21,3)*3]"  Inductances="[ line(21,4)  line(21,4)*3]"  Capacitances="[ line(21,5)  line(21,5)/3]"  Length=1
      settings: SourceProductName=Simscape Power Systems
  L-22 : powerlib/Elements/Three-Phase PI Section Line  LConnTagsString=a|b|c  RConnTagsString=A|B|C  Frequency=50  Resistances="[ line(22,3)  line(22,3)*3]"  Inductances="[ line(22,4)  line(22,4)*3]"  Capacitances="[ line(22,5)  line(22,5)/3]"  Length=1
      settings: SourceProductName=Simscape Power Systems
  L-23 : powerlib/Elements/Three-Phase PI Section Line  LConnTagsString=a|b|c  RConnTagsString=A|B|C  Frequency=50  Resistances="[ line(23,3)  line(23,3)*3]"  Inductances="[ line(23,4)  line(23,4)*3]"  Capacitances="[ line(23,5)  line(23,5)/3]"  Length=1
      settings: SourceProductName=Simscape Power Systems
  L-24-1 : powerlib/Elements/Three-Phase PI Section Line  LConnTagsString=a|b|c  RConnTagsString=A|B|C  Frequency=50  Resistances="[ line(24,3)  line(24,3)*3]"  Inductances="[ line(24,4)  line(24,4)*3]"  Capacitances="[ line(24,5)  line(24,5)/3]"  Length=1
      settings: SourceProductName=Simscape Power Systems
  L-24-2 : powerlib/Elements/Three-Phase PI Section Line  LConnTagsString=a|b|c  RConnTagsString=A|B|C  Frequency=50  Resistances="[ line(24,3)  line(24,3)*3]"  Inductances="[ line(24,4)  line(24,4)*3]"  Capacitances="[ line(24,5)  line(24,5)/3]"  Length=1
      settings: SourceProductName=Simscape Power Systems
  L-25 : powerlib/Elements/Three-Phase PI Section Line  LConnTagsString=a|b|c  RConnTagsString=A|B|C  Frequency=50  Resistances="[ line(25,3)  line(25,3)*3]"  Inductances="[ line(25,4)  line(25,4)*3]"  Capacitances="[ line(25,5)  line(25,5)/3]"  Length=1
      settings: SourceProductName=Simscape Power Systems
  L-26 : powerlib/Elements/Three-Phase PI Section Line  LConnTagsString=a|b|c  RConnTagsString=A|B|C  Frequency=50  Resistances="[ line(26,3)  line(26,3)*3]"  Inductances="[ line(26,4)  line(26,4)*3]"  Capacitances="[ line(26,5)  line(26,5)/3]"  Length=1
      settings: SourceProductName=Simscape Power Systems
  L-27-1 : powerlib/Elements/Three-Phase PI Section Line  LConnTagsString=a|b|c  RConnTagsString=A|B|C  Frequency=50  Resistances="[ line(27,3)  line(27,3)*3]"  Inductances="[ line(27,4)  line(27,4)*3]"  Capacitances="[ line(27,5)  line(27,5)/3]"  Length=1
      settings: SourceProductName=Simscape Power Systems
  L-27-2 : powerlib/Elements/Three-Phase PI Section Line  LConnTagsString=a|b|c  RConnTagsString=A|B|C  Frequency=50  Resistances="[ line(27,3)  line(27,3)*3]"  Inductances="[ line(27,4)  line(27,4)*3]"  Capacitances="[ line(27,5)  line(27,5)/3]"  Length=1
      settings: SourceProductName=Simscape Power Systems
  L-28 : powerlib/Elements/Three-Phase PI Section Line  LConnTagsString=a|b|c  RConnTagsString=A|B|C  Frequency=50  Resistances="[ line(28,3)  line(28,3)*3]"  Inductances="[ line(28,4)  line(28,4)*3]"  Capacitances="[ line(28,5)  line(28,5)/3]"  Length=1
      settings: SourceProductName=Simscape Power Systems
  L-29-1 : powerlib/Elements/Three-Phase PI Section Line  LConnTagsString=a|b|c  RConnTagsString=A|B|C  Frequency=50  Resistances="[ line(29,3)  line(29,3)*3]"  Inductances="[ line(29,4)  line(29,4)*3]"  Capacitances="[ line(29,5)  line(29,5)/3]"  Length=1
      settings: SourceProductName=Simscape Power Systems
  L-29-2 : powerlib/Elements/Three-Phase PI Section Line  LConnTagsString=a|b|c  RConnTagsString=A|B|C  Frequency=50  Resistances="[ line(29,3)  line(29,3)*3]"  Inductances="[ line(29,4)  line(29,4)*3]"  Capacitances="[ line(29,5)  line(29,5)/3]"  Length=1
      settings: SourceProductName=Simscape Power Systems
  L-3-1 : powerlib/Elements/Three-Phase PI Section Line  LConnTagsString=a|b|c  RConnTagsString=A|B|C  Frequency=50  Resistances="[ line(3,3)  line(3,3)*3]"  Inductances="[ line(3,4)  line(3,4)*3]"  Capacitances="[ line(3,5)  line(3,5)/3]"  Length=1
      settings: SourceProductName=Simscape Power Systems
  L-3-2 : powerlib/Elements/Three-Phase PI Section Line  LConnTagsString=a|b|c  RConnTagsString=A|B|C  Frequency=50  Resistances="[ line(3,3)  line(3,3)*3]"  Inductances="[ line(3,4)  line(3,4)*3]"  Capacitances="[ line(3,5)  line(3,5)/3]"  Length=1
      settings: SourceProductName=Simscape Power Systems
  L-30-1 : powerlib/Elements/Three-Phase PI Section Line  LConnTagsString=a|b|c  RConnTagsString=A|B|C  Frequency=50  Resistances="[ line(30,3)  line(30,3)*3]"  Inductances="[ line(30,4)  line(30,4)*3]"  Capacitances="[ line(30,5)  line(30,5)/3]"  Length=1
      settings: SourceProductName=Simscape Power Systems
  L-30-2 : powerlib/Elements/Three-Phase PI Section Line  LConnTagsString=a|b|c  RConnTagsString=A|B|C  Frequency=50  Resistances="[ line(30,3)  line(30,3)*3]"  Inductances="[ line(30,4)  line(30,4)*3]"  Capacitances="[ line(30,5)  line(30,5)/3]"  Length=1
      settings: SourceProductName=Simscape Power Systems
  L-32 : powerlib/Elements/Three-Phase PI Section Line  LConnTagsString=a|b|c  RConnTagsString=A|B|C  Frequency=50  Resistances="[ line(32,3)  line(32,3)*3]"  Inductances="[ line(32,4)  line(32,4)*3]"  Capacitances="[ line(32,5)  line(32,5)/3]"  Length=1
      settings: SourceProductName=Simscape Power Systems
  L-33 : powerlib/Elements/Three-Phase PI Section Line  LConnTagsString=a|b|c  RConnTagsString=A|B|C  Frequency=50  Resistances="[ line(33,3)  line(33,3)*3]"  Inductances="[ line(33,4)  line(33,4)*3]"  Capacitances="[ line(33,5)  line(33,5)/3]"  Length=1
      settings: SourceProductName=Simscape Power Systems
  L-34-1 : powerlib/Elements/Three-Phase PI Section Line  LConnTagsString=a|b|c  RConnTagsString=A|B|C  Frequency=50  Resistances="[ line(34,3)  line(34,3)*3]"  Inductances="[ line(34,4)  line(34,4)*3]"  Capacitances="[ line(34,5)  line(34,5)/3]"  Length=1
      settings: SourceProductName=Simscape Power Systems
  L-34-2 : powerlib/Elements/Three-Phase PI Section Line  LConnTagsString=a|b|c  RConnTagsString=A|B|C  Frequency=50  Resistances="[ line(34,3)  line(34,3)*3]"  Inductances="[ line(34,4)  line(34,4)*3]"  Capacitances="[ line(34,5)  line(34,5)/3]"  Length=1
      settings: SourceProductName=Simscape Power Systems
  L-35-1 : powerlib/Elements/Three-Phase PI Section Line  LConnTagsString=a|b|c  RConnTagsString=A|B|C  Frequency=50  Resistances="[ line(35,3)  line(35,3)*3]"  Inductances="[ line(35,4)  line(35,4)*3]"  Capacitances="[ line(35,5)  line(35,5)/3]"  Length=1
      settings: SourceProductName=Simscape Power Systems
  L-35-2 : powerlib/Elements/Three-Phase PI Section Line  LConnTagsString=a|b|c  RConnTagsString=A|B|C  Frequency=50  Resistances="[ line(35,3)  line(35,3)*3]"  Inductances="[ line(35,4)  line(35,4)*3]"  Capacitances="[ line(35,5)  line(35,5)/3]"  Length=1
      settings: SourceProductName=Simscape Power Systems
  L-36-1 : powerlib/Elements/Three-Phase PI Section Line  LConnTagsString=a|b|c  RConnTagsString=A|B|C  Frequency=50  Resistances="[ line(36,3)  line(36,3)*3]"  Inductances="[ line(36,4)  line(36,4)*3]"  Capacitances="[ line(36,5)  line(36,5)/3]"  Length=1
      settings: SourceProductName=Simscape Power Systems
  L-37-1 : powerlib/Elements/Three-Phase PI Section Line  LConnTagsString=a|b|c  RConnTagsString=A|B|C  Frequency=50  Resistances="[ line(37,3)  line(37,3)*3]"  Inductances="[ line(37,4)  line(37,4)*3]"  Capacitances="[ line(37,5)  line(37,5)/3]"  Length=1
      settings: SourceProductName=Simscape Power Systems
  L-37-2 : powerlib/Elements/Three-Phase PI Section Line  LConnTagsString=a|b|c  RConnTagsString=A|B|C  Frequency=50  Resistances="[ line(37,3)  line(37,3)*3]"  Inductances="[ line(37,4)  line(37,4)*3]"  Capacitances="[ line(37,5)  line(37,5)/3]"  Length=1
      settings: SourceProductName=Simscape Power Systems
  L-37-3 : powerlib/Elements/Three-Phase PI Section Line  LConnTagsString=a|b|c  RConnTagsString=A|B|C  Frequency=50  Resistances="[ line(37,3)  line(37,3)*3]"  Inductances="[ line(37,4)  line(37,4)*3]"  Capacitances="[ line(37,5)  line(37,5)/3]"  Length=1
      settings: SourceProductName=Simscape Power Systems
  L-38-1 : powerlib/Elements/Three-Phase PI Section Line  LConnTagsString=a|b|c  RConnTagsString=A|B|C  Frequency=50  Resistances="[ line(38,3)  line(38,3)*3]"  Inductances="[ line(38,4)  line(38,4)*3]"  Capacitances="[ line(38,5)  line(38,5)/3]"  Length=1
      settings: SourceProductName=Simscape Power Systems
  L-38-2 : powerlib/Elements/Three-Phase PI Section Line  LConnTagsString=a|b|c  RConnTagsString=A|B|C  Frequency=50  Resistances="[ line(38,3)  line(38,3)*3]"  Inductances="[ line(38,4)  line(38,4)*3]"  Capacitances="[ line(38,5)  line(38,5)/3]"  Length=1
      settings: SourceProductName=Simscape Power Systems
  L-39 : powerlib/Elements/Three-Phase PI Section Line  LConnTagsString=a|b|c  RConnTagsString=A|B|C  Frequency=50  Resistances="[ line(39,3)  line(39,3)*3]"  Inductances="[ line(39,4)  line(39,4)*3]"  Capacitances="[ line(39,5)  line(39,5)/3]"  Length=1
      settings: SourceProductName=Simscape Power Systems
  L-4 : powerlib/Elements/Three-Phase PI Section Line  LConnTagsString=a|b|c  RConnTagsString=A|B|C  Frequency=50  Resistances="[ line(4,3)  line(4,3)*3]"  Inductances="[ line(4,4)  line(4,4)*3]"  Capacitances="[ line(4,5)  line(4,5)/3]"  Length=1
      settings: SourceProductName=Simscape Power Systems
  L-40-1 : powerlib/Elements/Three-Phase PI Section Line  LConnTagsString=a|b|c  RConnTagsString=A|B|C  Frequency=50  Resistances="[ line(40,3)  line(40,3)*3]"  Inductances="[ line(40,4)  line(40,4)*3]"  Capacitances="[ line(40,5)  line(40,5)/3]"  Length=1
      settings: SourceProductName=Simscape Power Systems
  L-40-2 : powerlib/Elements/Three-Phase PI Section Line  LConnTagsString=a|b|c  RConnTagsString=A|B|C  Frequency=50  Resistances="[ line(40,3)  line(40,3)*3]"  Inductances="[ line(40,4)  line(40,4)*3]"  Capacitances="[ line(40,5)  line(40,5)/3]"  Length=1
      settings: SourceProductName=Simscape Power Systems
  L-41-1 : powerlib/Elements/Three-Phase PI Section Line  LConnTagsString=a|b|c  RConnTagsString=A|B|C  Frequency=50  Resistances="[ line(41,3)  line(41,3)*3]"  Inductances="[ line(41,4)  line(41,4)*3]"  Capacitances="[ line(41,5)  line(41,5)/3]"  Length=1
      settings: SourceProductName=Simscape Power Systems
  L-41-2 : powerlib/Elements/Three-Phase PI Section Line  LConnTagsString=a|b|c  RConnTagsString=A|B|C  Frequency=50  Resistances="[ line(41,3)  line(41,3)*3]"  Inductances="[ line(41,4)  line(41,4)*3]"  Capacitances="[ line(41,5)  line(41,5)/3]"  Length=1
      settings: SourceProductName=Simscape Power Systems
  L-42 : powerlib/Elements/Three-Phase PI Section Line  LConnTagsString=a|b|c  RConnTagsString=A|B|C  Frequency=50  Resistances="[ line(42,3)  line(42,3)*3]"  Inductances="[ line(42,4)  line(42,4)*3]"  Capacitances="[ line(42,5)  line(42,5)/3]"  Length=1
      settings: SourceProductName=Simscape Power Systems
  L-43-{1..4} (4 alike) : powerlib/Elements/Three-Phase PI Section Line  LConnTagsString=a|b|c  RConnTagsString=A|B|C  Frequency=50  Resistances="[ line(43,3)  line(43,3)*3]"  Inductances="[ line(43,4)  line(43,4)*3]"  Capacitances="[ line(43,5)  line(43,5)/3]"  Length=1
      settings: SourceProductName=Simscape Power Systems
  L-44-1 : powerlib/Elements/Three-Phase PI Section Line  LConnTagsString=a|b|c  RConnTagsString=A|B|C  Frequency=50  Resistances="[ line(44,3)  line(44,3)*3]"  Inductances="[ line(44,4)  line(44,4)*3]"  Capacitances="[ line(44,5)  line(44,5)/3]"  Length=1
      settings: SourceProductName=Simscape Power Systems
  L-44-2 : powerlib/Elements/Three-Phase PI Section Line  LConnTagsString=a|b|c  RConnTagsString=A|B|C  Frequency=50  Resistances="[ line(44,3)  line(44,3)*3]"  Inductances="[ line(44,4)  line(44,4)*3]"  Capacitances="[ line(44,5)  line(44,5)/3]"  Length=1
      settings: SourceProductName=Simscape Power Systems
  L-45-1 : powerlib/Elements/Three-Phase PI Section Line  LConnTagsString=a|b|c  RConnTagsString=A|B|C  Frequency=50  Resistances="[ line(45,3)  line(45,3)*3]"  Inductances="[ line(45,4)  line(45,4)*3]"  Capacitances="[ line(45,5)  line(45,5)/3]"  Length=1
      settings: SourceProductName=Simscape Power Systems
  L-45-2 : powerlib/Elements/Three-Phase PI Section Line  LConnTagsString=a|b|c  RConnTagsString=A|B|C  Frequency=50  Resistances="[ line(45,3)  line(45,3)*3]"  Inductances="[ line(45,4)  line(45,4)*3]"  Capacitances="[ line(45,5)  line(45,5)/3]"  Length=1
      settings: SourceProductName=Simscape Power Systems
  L-46-1 : powerlib/Elements/Three-Phase PI Section Line  LConnTagsString=a|b|c  RConnTagsString=A|B|C  Frequency=50  Resistances="[ line(46,3)  line(46,3)*3]"  Inductances="[ line(46,4)  line(46,4)*3]"  Capacitances="[ line(46,5)  line(46,5)/3]"  Length=1
      settings: SourceProductName=Simscape Power Systems
  L-46-2 : powerlib/Elements/Three-Phase PI Section Line  LConnTagsString=a|b|c  RConnTagsString=A|B|C  Frequency=50  Resistances="[ line(46,3)  line(46,3)*3]"  Inductances="[ line(46,4)  line(46,4)*3]"  Capacitances="[ line(46,5)  line(46,5)/3]"  Length=1
      settings: SourceProductName=Simscape Power Systems
  L-47-1 : powerlib/Elements/Three-Phase PI Section Line  LConnTagsString=a|b|c  RConnTagsString=A|B|C  Frequency=50  Resistances="[ line(47,3)  line(47,3)*3]"  Inductances="[ line(47,4)  line(47,4)*3]"  Capacitances="[ line(47,5)  line(47,5)/3]"  Length=1
      settings: SourceProductName=Simscape Power Systems
  L-47-2 : powerlib/Elements/Three-Phase PI Section Line  LConnTagsString=a|b|c  RConnTagsString=A|B|C  Frequency=50  Resistances="[ line(47,3)  line(47,3)*3]"  Inductances="[ line(47,4)  line(47,4)*3]"  Capacitances="[ line(47,5)  line(47,5)/3]"  Length=1
      settings: SourceProductName=Simscape Power Systems
  L-48-1 : powerlib/Elements/Three-Phase PI Section Line  LConnTagsString=a|b|c  RConnTagsString=A|B|C  Frequency=50  Resistances="[ line(48,3)  line(48,3)*3]"  Inductances="[ line(48,4)  line(48,4)*3]"  Capacitances="[ line(48,5)  line(48,5)/3]"  Length=1
      settings: SourceProductName=Simscape Power Systems
  L-48-2 : powerlib/Elements/Three-Phase PI Section Line  LConnTagsString=a|b|c  RConnTagsString=A|B|C  Frequency=50  Resistances="[ line(48,3)  line(48,3)*3]"  Inductances="[ line(48,4)  line(48,4)*3]"  Capacitances="[ line(48,5)  line(48,5)/3]"  Length=1
      settings: SourceProductName=Simscape Power Systems
  L-49-1 : powerlib/Elements/Three-Phase PI Section Line  LConnTagsString=a|b|c  RConnTagsString=A|B|C  Frequency=50  Resistances="[ line(49,3)  line(49,3)*3]"  Inductances="[ line(49,4)  line(49,4)*3]"  Capacitances="[ line(49,5)  line(49,5)/3]"  Length=1
      settings: SourceProductName=Simscape Power Systems
  L-49-2 : powerlib/Elements/Three-Phase PI Section Line  LConnTagsString=a|b|c  RConnTagsString=A|B|C  Frequency=50  Resistances="[ line(49,3)  line(49,3)*3]"  Inductances="[ line(49,4)  line(49,4)*3]"  Capacitances="[ line(49,5)  line(49,5)/3]"  Length=1
      settings: SourceProductName=Simscape Power Systems
  L-5-1 : powerlib/Elements/Three-Phase PI Section Line  LConnTagsString=a|b|c  RConnTagsString=A|B|C  Frequency=50  Resistances="[ line(5,3)  line(5,3)*3]"  Inductances="[ line(5,4)  line(5,4)*3]"  Capacitances="[ line(5,5)  line(5,5)/3]"  Length=1
      settings: SourceProductName=Simscape Power Systems
  L-5-2 : powerlib/Elements/Three-Phase PI Section Line  LConnTagsString=a|b|c  RConnTagsString=A|B|C  Frequency=50  Resistances="[ line(5,3)  line(5,3)*3]"  Inductances="[ line(5,4)  line(5,4)*3]"  Capacitances="[ line(5,5)  line(5,5)/3]"  Length=1
      settings: SourceProductName=Simscape Power Systems
  L-50-1 : powerlib/Elements/Three-Phase PI Section Line  LConnTagsString=a|b|c  RConnTagsString=A|B|C  Frequency=50  Resistances="[ line(50,3)  line(50,3)*3]"  Inductances="[ line(50,4)  line(50,4)*3]"  Capacitances="[ line(50,5)  line(50,5)/3]"  Length=1
      settings: SourceProductName=Simscape Power Systems
  L-51 : powerlib/Elements/Three-Phase PI Section Line  LConnTagsString=a|b|c  RConnTagsString=A|B|C  Frequency=50  Resistances="[ line(51,3)  line(51,3)*3]"  Inductances="[ line(51,4)  line(51,4)*3]"  Capacitances="[ line(51,5)  line(51,5)/3]"  Length=1
      settings: SourceProductName=Simscape Power Systems
  L-52 : powerlib/Elements/Three-Phase PI Section Line  LConnTagsString=a|b|c  RConnTagsString=A|B|C  Frequency=50  Resistances="[ line(52,3)  line(52,3)*3]"  Inductances="[ line(52,4)  line(52,4)*3]"  Capacitances="[ line(52,5)  line(52,5)/3]"  Length=1
      settings: SourceProductName=Simscape Power Systems
  L-53 : powerlib/Elements/Three-Phase PI Section Line  LConnTagsString=a|b|c  RConnTagsString=A|B|C  Frequency=50  Resistances="[ line(53,3)  line(53,3)*3]"  Inductances="[ line(53,4)  line(53,4)*3]"  Capacitances="[ line(53,5)  line(53,5)/3]"  Length=1
      settings: SourceProductName=Simscape Power Systems
  L-54 : powerlib/Elements/Three-Phase PI Section Line  LConnTagsString=a|b|c  RConnTagsString=A|B|C  Frequency=50  Resistances=[ line(54,3) line(54,3)*3]  Inductances=[ line(54,4) line(54,4)*3]  Capacitances=[ line(54,5) line(54,5)/3]  Length=1
      settings: SourceProductName=Simscape Power Systems
  L-55-1 : powerlib/Elements/Three-Phase PI Section Line  LConnTagsString=a|b|c  RConnTagsString=A|B|C  Frequency=50  Resistances=[ line(55,3) line(55,3)*3]  Inductances="[ line(55,4)  line(55,4)*3]"  Capacitances="[line(55,5)  line(55,5)/3]"  Length=1
      settings: SourceProductName=Simscape Power Systems
  L-55-2 : powerlib/Elements/Three-Phase PI Section Line  LConnTagsString=a|b|c  RConnTagsString=A|B|C  Frequency=50  Resistances=[ line(55,3) line(55,3)*3]  Inductances="[ line(55,4)  line(55,4)*3]"  Capacitances="[line(55,5)  line(55,5)/3]"  Length=1
      settings: SourceProductName=Simscape Power Systems
  L-6-1 : powerlib/Elements/Three-Phase PI Section Line  LConnTagsString=a|b|c  RConnTagsString=A|B|C  Frequency=50  Resistances="[ line(6,3)  line(6,3)*3]"  Inductances="[ line(6,4)  line(6,4)*3]"  Capacitances="[ line(6,5)  line(6,5)/3]"  Length=1
      settings: SourceProductName=Simscape Power Systems
  L-6-2 : powerlib/Elements/Three-Phase PI Section Line  LConnTagsString=a|b|c  RConnTagsString=A|B|C  Frequency=50  Resistances="[ line(6,3)  line(6,3)*3]"  Inductances="[ line(6,4)  line(6,4)*3]"  Capacitances="[ line(6,5)  line(6,5)/3]"  Length=1
      settings: SourceProductName=Simscape Power Systems
  L-7-1 : powerlib/Elements/Three-Phase PI Section Line  LConnTagsString=a|b|c  RConnTagsString=A|B|C  Frequency=50  Resistances="[ line(7,3)  line(7,3)*3]"  Inductances="[ line(7,4)  line(7,4)*3]"  Capacitances="[ line(7,5)  line(7,5)/3]"  Length=1
      settings: SourceProductName=Simscape Power Systems
  L-7-2 : powerlib/Elements/Three-Phase PI Section Line  LConnTagsString=a|b|c  RConnTagsString=A|B|C  Frequency=50  Resistances="[ line(7,3)  line(7,3)*3]"  Inductances="[ line(7,4)  line(7,4)*3]"  Capacitances="[ line(7,5)  line(7,5)/3]"  Length=1
      settings: SourceProductName=Simscape Power Systems
  L-8-1 : powerlib/Elements/Three-Phase PI Section Line  LConnTagsString=a|b|c  RConnTagsString=A|B|C  Frequency=50  Resistances="[ line(8,3)  line(8,3)*3]"  Inductances="[ line(8,4)  line(8,4)*3]"  Capacitances="[ line(8,5)  line(8,5)/3]"  Length=1
      settings: SourceProductName=Simscape Power Systems
  L-8-2 : powerlib/Elements/Three-Phase PI Section Line  LConnTagsString=a|b|c  RConnTagsString=A|B|C  Frequency=50  Resistances="[ line(8,3)  line(8,3)*3]"  Inductances="[ line(8,4)  line(8,4)*3]"  Capacitances="[ line(8,5)  line(8,5)/3]"  Length=1
      settings: SourceProductName=Simscape Power Systems
  L-9-1 : powerlib/Elements/Three-Phase PI Section Line  LConnTagsString=a|b|c  RConnTagsString=A|B|C  Frequency=50  Resistances="[ line(9,3)  line(9,3)*3]"  Inductances="[ line(9,4)  line(9,4)*3]"  Capacitances="[ line(9,5)  line(9,5)/3]"  Length=1
      settings: SourceProductName=Simscape Power Systems
  L-9-2 : powerlib/Elements/Three-Phase PI Section Line  LConnTagsString=a|b|c  RConnTagsString=A|B|C  Frequency=50  Resistances="[ line(9,3)  line(9,3)*3]"  Inductances="[ line(9,4)  line(9,4)*3]"  Capacitances="[ line(9,5)  line(9,5)/3]"  Length=1
      settings: SourceProductName=Simscape Power Systems
  LPS_3 : Subsystem
  Load Flow Bus1 : powerlib/Measurements/Load Flow Bus  LConnTagsString=a  Phases=single  Connectors=on one side  ID=B403  Vbase=20e3  Vref=1  Vangle=0  VLF=1  VLFb=1  VLFc=1  angleLF=0.3283  angleLFb=0  angleLFc=0
      settings: AttributesFormatString=%<ID>\n%<Vbase>V\n%<VLF>pu\n%<angleLF>deg.  SourceProductName=Simscape Power Systems
  Load Flow Bus10 : powerlib/Measurements/Load Flow Bus  LConnTagsString=a  Phases=single  Connectors=on one side  ID=B301  Vbase=20e3  Vref=1  Vangle=0  VLF=1  VLFb=1  VLFc=1  angleLF=-8.535  angleLFb=0  angleLFc=0
      settings: AttributesFormatString=%<ID>\n%<Vbase>V\n%<VLF>pu\n%<angleLF>deg.  SourceProductName=Simscape Power Systems
  Load Flow Bus11 : powerlib/Measurements/Load Flow Bus  LConnTagsString=a  Phases=single  Connectors=on one side  ID=B302  Vbase=20e3  Vref=1  Vangle=0  VLF=1  VLFb=1  VLFc=1  angleLF=-17.5  angleLFb=0  angleLFc=0
      settings: AttributesFormatString=%<ID>\n%<Vbase>V\n%<VLF>pu\n%<angleLF>deg.  SourceProductName=Simscape Power Systems
  Load Flow Bus12 : powerlib/Measurements/Load Flow Bus  LConnTagsString=a  Phases=single  Connectors=on one side  ID=B503  Vbase=15e3  Vref=1  Vangle=0  VLF=1  VLFb=1  VLFc=1  angleLF=-36.71  angleLFb=0  angleLFc=0
      settings: AttributesFormatString=%<ID>\n%<Vbase>V\n%<VLF>pu\n%<angleLF>deg.  SourceProductName=Simscape Power Systems
  Load Flow Bus13 : powerlib/Measurements/Load Flow Bus  LConnTagsString=a  Phases=single  Connectors=on one side  ID=B502  Vbase=15e3  Vref=1  Vangle=0  VLF=1  VLFb=1  VLFc=1  angleLF=-31.12  angleLFb=0  angleLFc=0
      settings: AttributesFormatString=%<ID>\n%<Vbase>V\n%<VLF>pu\n%<angleLF>deg.  SourceProductName=Simscape Power Systems
  Load Flow Bus14 : powerlib/Measurements/Load Flow Bus  LConnTagsString=a  Phases=single  Connectors=on one side  ID=B501  Vbase=20e3  Vref=1  Vangle=0  VLF=1  VLFb=1  VLFc=1  angleLF=-32.78  angleLFb=0  angleLFc=0
      settings: AttributesFormatString=%<ID>\n%<Vbase>V\n%<VLF>pu\n%<angleLF>deg.  SourceProductName=Simscape Power Systems
  Load Flow Bus2 : powerlib/Measurements/Load Flow Bus  LConnTagsString=a  Phases=single  Connectors=on one side  ID=B404  Vbase=20e3  Vref=1  Vangle=0  VLF=1  VLFb=1  VLFc=1  angleLF=-6.285  angleLFb=0  angleLFc=0
      settings: AttributesFormatString=%<ID>\n%<Vbase>V\n%<VLF>pu\n%<angleLF>deg.  SourceProductName=Simscape Power Systems
  Load Flow Bus3 : powerlib/Measurements/Load Flow Bus  LConnTagsString=a  Phases=single  Connectors=on one side  ID=B402  Vbase=20e3  Vref=1  Vangle=0  VLF=1  VLFb=1  VLFc=1  angleLF=0.6296  angleLFb=0  angleLFc=0
      settings: AttributesFormatString=%<ID>\n%<Vbase>V\n%<VLF>pu\n%<angleLF>deg.  SourceProductName=Simscape Power Systems
  Load Flow Bus4 : powerlib/Measurements/Load Flow Bus  LConnTagsString=a  Phases=single  Connectors=on one side  ID=B401  Vbase=20e3  Vref=1  Vangle=0  VLF=1  VLFb=1  VLFc=1  angleLF=-14.29  angleLFb=0  angleLFc=0
      settings: AttributesFormatString=%<ID>\n%<Vbase>V\n%<VLF>pu\n%<angleLF>deg.  SourceProductName=Simscape Power Systems
  Load Flow Bus5 : powerlib/Measurements/Load Flow Bus  LConnTagsString=a  Phases=single  Connectors=on one side  ID=B203  Vbase=20e3  Vref=1  Vangle=0  VLF=1  VLFb=1  VLFc=1  angleLF=0.6457  angleLFb=0  angleLFc=0
      settings: AttributesFormatString=%<ID>\n%<Vbase>V\n%<VLF>pu\n%<angleLF>deg.  SourceProductName=Simscape Power Systems
  Load Flow Bus6 : powerlib/Measurements/Load Flow Bus  LConnTagsString=a  Phases=single  Connectors=on one side  ID=B201  Vbase=20e3  Vref=1  Vangle=0  VLF=1  VLFb=1  VLFc=1  angleLF=5.269  angleLFb=0  angleLFc=0
      settings: AttributesFormatString=%<ID>\n%<Vbase>V\n%<VLF>pu\n%<angleLF>deg.  SourceProductName=Simscape Power Systems
  Load Flow Bus7 : powerlib/Measurements/Load Flow Bus  LConnTagsString=a  Phases=single  Connectors=on one side  ID=B202  Vbase=20e3  Vref=1  Vangle=0  VLF=1  VLFb=1  VLFc=1  angleLF=0.9722  angleLFb=0  angleLFc=0
      settings: AttributesFormatString=%<ID>\n%<Vbase>V\n%<VLF>pu\n%<angleLF>deg.  SourceProductName=Simscape Power Systems
  Load Flow Bus8 : powerlib/Measurements/Load Flow Bus  LConnTagsString=a  Phases=single  Connectors=on one side  ID=B204  Vbase=20e3  Vref=1  Vangle=0  VLF=1  VLFb=1  VLFc=1  angleLF=0  angleLFb=0  angleLFc=0
      settings: AttributesFormatString=%<ID>\n%<Vbase>V\n%<VLF>pu\n%<angleLF>deg.  SourceProductName=Simscape Power Systems
  Load Flow Bus9 : powerlib/Measurements/Load Flow Bus  LConnTagsString=a  Phases=single  Connectors=on one side  ID=B101  Vbase=15e3  Vref=1  Vangle=0  VLF=1  VLFb=1  VLFc=1  angleLF=-22.34  angleLFb=0  angleLFc=0
      settings: AttributesFormatString=%<ID>\n%<Vbase>V\n%<VLF>pu\n%<angleLF>deg.  SourceProductName=Simscape Power Systems
  Load1 : powerlib/Elements/Three-Phase Parallel RLC Load  LConnTagsString=A|B|C  Configuration=Y (grounded)  NominalVoltage=(342408)*1.00042  Vabc=[1e3 1e3 1e3]  Vabcp=[1e3 1e3 1e3]  NominalFrequency=50  UnbalancedPower=off  ActivePower=load(1,2)*1e6  InductivePower=load(1,3)*1e6  CapacitivePower=0  Pabc=[10e3 9e3 11e3]  QLabc=[100 90 110]  QCabc=[100 90 110]  Pabcp=[10e3 9e3 11e3]  QLabcp=[100 90 110]  QCabcp=[100 90 110]  Measurements=None  LoadType=constant PQ
  Load10 : powerlib/Elements/Three-Phase Parallel RLC Load  LConnTagsString=A|B|C  Configuration=Y (grounded)  NominalVoltage=(339983)*1.00045  Vabc=[1e3 1e3 1e3]  Vabcp=[1e3 1e3 1e3]  NominalFrequency=50  UnbalancedPower=off  ActivePower=load(10,2)*1e6  InductivePower=load(10,3)*1e6  CapacitivePower=0  Pabc=[10e3 9e3 11e3]  QLabc=[100 90 110]  QCabc=[100 90 110]  Pabcp=[10e3 9e3 11e3]  QLabcp=[100 90 110]  QCabcp=[100 90 110]  Measurements=None  LoadType=constant PQ
  Load11 : powerlib/Elements/Three-Phase Parallel RLC Load  LConnTagsString=A|B|C  Configuration=Y (grounded)  NominalVoltage=(508840)*1.00261  Vabc=[1e3 1e3 1e3]  Vabcp=[1e3 1e3 1e3]  NominalFrequency=50  UnbalancedPower=off  ActivePower=load(11,2)*1e6  InductivePower=load(11,3)*1e6  CapacitivePower=0  Pabc=[10e3 9e3 11e3]  QLabc=[100 90 110]  QCabc=[100 90 110]  Pabcp=[10e3 9e3 11e3]  QLabcp=[100 90 110]  QCabcp=[100 90 110]  Measurements=None  LoadType=constant PQ
  Load12 : powerlib/Elements/Three-Phase Parallel RLC Load  LConnTagsString=A|B|C  Configuration=Y (grounded)  NominalVoltage=(510075)*1.00296  Vabc=[1e3 1e3 1e3]  Vabcp=[1e3 1e3 1e3]  NominalFrequency=50  UnbalancedPower=off  ActivePower=load(12,2)*1e6  InductivePower=load(12,3)*1e6  CapacitivePower=0  Pabc=[10e3 9e3 11e3]  QLabc=[100 90 110]  QCabc=[100 90 110]  Pabcp=[10e3 9e3 11e3]  QLabcp=[100 90 110]  QCabcp=[100 90 110]  Measurements=None  LoadType=constant PQ
  Load13 : powerlib/Elements/Three-Phase Parallel RLC Load  LConnTagsString=A|B|C  Configuration=Y (grounded)  NominalVoltage=(521840)*1.01599  Vabc=[1e3 1e3 1e3]  Vabcp=[1e3 1e3 1e3]  NominalFrequency=50  UnbalancedPower=off  ActivePower=load(13,2)*1e6  InductivePower=load(13,3)*1e6  CapacitivePower=0  Pabc=[10e3 9e3 11e3]  QLabc=[100 90 110]  QCabc=[100 90 110]  Pabcp=[10e3 9e3 11e3]  QLabcp=[100 90 110]  QCabcp=[100 90 110]  Measurements=None  LoadType=constant PQ
  Load14 : powerlib/Elements/Three-Phase Parallel RLC Load  LConnTagsString=A|B|C  Configuration=Y (grounded)  NominalVoltage=(346731)*1.00073  Vabc=[1e3 1e3 1e3]  Vabcp=[1e3 1e3 1e3]  NominalFrequency=50  UnbalancedPower=off  ActivePower=load(14,2)*1e6  InductivePower=load(14,3)*1e6  CapacitivePower=0  Pabc=[10e3 9e3 11e3]  QLabc=[100 90 110]  QCabc=[100 90 110]  Pabcp=[10e3 9e3 11e3]  QLabcp=[100 90 110]  QCabcp=[100 90 110]  Measurements=None  LoadType=constant PQ
  Load15 : powerlib/Elements/Three-Phase Parallel RLC Load  LConnTagsString=A|B|C  Configuration=Y (grounded)  NominalVoltage=(220647)*0.997322  Vabc=[1e3 1e3 1e3]  Vabcp=[1e3 1e3 1e3]  NominalFrequency=50  UnbalancedPower=off  ActivePower=load(15,2)*1e6  InductivePower=load(15,3)*1e6  CapacitivePower=0  Pabc=[10e3 9e3 11e3]  QLabc=[100 90 110]  QCabc=[100 90 110]  Pabcp=[10e3 9e3 11e3]  QLabcp=[100 90 110]  QCabcp=[100 90 110]  Measurements=None  LoadType=constant PQ
  Load16 : powerlib/Elements/Three-Phase Parallel RLC Load  LConnTagsString=A|B|C  Configuration=Y (grounded)  NominalVoltage=(219851)*0.994974  Vabc=[1e3 1e3 1e3]  Vabcp=[1e3 1e3 1e3]  NominalFrequency=50  UnbalancedPower=off  ActivePower=load(16,2)*1e6  InductivePower=load(16,3)*1e6  CapacitivePower=0  Pabc=[10e3 9e3 11e3]  QLabc=[100 90 110]  QCabc=[100 90 110]  Pabcp=[10e3 9e3 11e3]  QLabcp=[100 90 110]  QCabcp=[100 90 110]  Measurements=None  LoadType=constant PQ
  Load17 : powerlib/Elements/Three-Phase Parallel RLC Load  LConnTagsString=A|B|C  Configuration=Y (grounded)  NominalVoltage=(221063)*0.996965  Vabc=[1e3 1e3 1e3]  Vabcp=[1e3 1e3 1e3]  NominalFrequency=50  UnbalancedPower=off  ActivePower=load(17,2)*1e6  InductivePower=load(17,3)*1e6  CapacitivePower=0  Pabc=[10e3 9e3 11e3]  QLabc=[100 90 110]  QCabc=[100 90 110]  Pabcp=[10e3 9e3 11e3]  QLabcp=[100 90 110]  QCabcp=[100 90 110]  Measurements=None  LoadType=constant PQ
  Load18 : powerlib/Elements/Three-Phase Parallel RLC Load  LConnTagsString=A|B|C  Configuration=Y (grounded)  NominalVoltage=(277236)*1.00165  Vabc=[1e3 1e3 1e3]  Vabcp=[1e3 1e3 1e3]  NominalFrequency=50  UnbalancedPower=off  ActivePower=load(18,2)*1e6  InductivePower=load(18,3)*1e6  CapacitivePower=0  Pabc=[10e3 9e3 11e3]  QLabc=[100 90 110]  QCabc=[100 90 110]  Pabcp=[10e3 9e3 11e3]  QLabcp=[100 90 110]  QCabcp=[100 90 110]  Measurements=None  LoadType=constant PQ
  Load19 : powerlib/Elements/Three-Phase Parallel RLC Load  LConnTagsString=A|B|C  Configuration=Y (grounded)  NominalVoltage=(274845)*1.0008  Vabc=[1e3 1e3 1e3]  Vabcp=[1e3 1e3 1e3]  NominalFrequency=50  UnbalancedPower=off  ActivePower=load(19,2)*1e6  InductivePower=load(19,3)*1e6  CapacitivePower=0  Pabc=[10e3 9e3 11e3]  QLabc=[100 90 110]  QCabc=[100 90 110]  Pabcp=[10e3 9e3 11e3]  QLabcp=[100 90 110]  QCabcp=[100 90 110]  Measurements=None  LoadType=constant PQ
  Load2 : powerlib/Elements/Three-Phase Parallel RLC Load  LConnTagsString=A|B|C  Configuration=Y (grounded)  NominalVoltage=(345688)*1.01324  Vabc=[1e3 1e3 1e3]  Vabcp=[1e3 1e3 1e3]  NominalFrequency=50  UnbalancedPower=off  ActivePower=load(2,2)*1e6  InductivePower=load(2,3)*1e6  CapacitivePower=0  Pabc=[10e3 9e3 11e3]  QLabc=[100 90 110]  QCabc=[100 90 110]  Pabcp=[10e3 9e3 11e3]  QLabcp=[100 90 110]  QCabcp=[100 90 110]  Measurements=None  LoadType=constant PQ
  Load20 : powerlib/Elements/Three-Phase Parallel RLC Load  LConnTagsString=A|B|C  Configuration=Y (grounded)  NominalVoltage=(275322)*1.00065  Vabc=[1e3 1e3 1e3]  Vabcp=[1e3 1e3 1e3]  NominalFrequency=50  UnbalancedPower=off  ActivePower=load(20,2)*1e6  InductivePower=load(20,3)*1e6  CapacitivePower=0  Pabc=[10e3 9e3 11e3]  QLabc=[100 90 110]  QCabc=[100 90 110]  Pabcp=[10e3 9e3 11e3]  QLabcp=[100 90 110]  QCabcp=[100 90 110]  Measurements=None  LoadType=constant PQ
  Load21 : powerlib/Elements/Three-Phase Parallel RLC Load  LConnTagsString=A|B|C  Configuration=Y (grounded)  NominalVoltage=(278338)*1.00157  Vabc=[1e3 1e3 1e3]  Vabcp=[1e3 1e3 1e3]  NominalFrequency=50  UnbalancedPower=off  ActivePower=load(21,2)*1e6  InductivePower=load(21,3)*1e6  CapacitivePower=0  Pabc=[10e3 9e3 11e3]  QLabc=[100 90 110]  QCabc=[100 90 110]  Pabcp=[10e3 9e3 11e3]  QLabcp=[100 90 110]  QCabcp=[100 90 110]  Measurements=None  LoadType=constant PQ
  Load22 : powerlib/Elements/Three-Phase Parallel RLC Load  LConnTagsString=A|B|C  Configuration=Y (grounded)  NominalVoltage=(275000)*1.03987  Vabc=[1e3 1e3 1e3]  Vabcp=[1e3 1e3 1e3]  NominalFrequency=50  UnbalancedPower=off  ActivePower=load(22,2)*1e6  InductivePower=load(22,3)*1e6  CapacitivePower=0  Pabc=[10e3 9e3 11e3]  QLabc=[100 90 110]  QCabc=[100 90 110]  Pabcp=[10e3 9e3 11e3]  QLabcp=[100 90 110]  QCabcp=[100 90 110]  Measurements=None  LoadType=constant PQ
  Load23 : powerlib/Elements/Three-Phase Parallel RLC Load  LConnTagsString=A|B|C  Configuration=Y (grounded)  NominalVoltage=(278284)*1.00613  Vabc=[1e3 1e3 1e3]  Vabcp=[1e3 1e3 1e3]  NominalFrequency=50  UnbalancedPower=off  ActivePower=load(23,2)*1e6  InductivePower=load(23,3)*1e6  CapacitivePower=0  Pabc=[10e3 9e3 11e3]  QLabc=[100 90 110]  QCabc=[100 90 110]  Pabcp=[10e3 9e3 11e3]  QLabcp=[100 90 110]  QCabcp=[100 90 110]  Measurements=None  LoadType=constant PQ
  Load24 : powerlib/Elements/Three-Phase Parallel RLC Load  LConnTagsString=A|B|C  Configuration=Y (grounded)  NominalVoltage=(275000)*1.01609  Vabc=[1e3 1e3 1e3]  Vabcp=[1e3 1e3 1e3]  NominalFrequency=50  UnbalancedPower=off  ActivePower=load(24,2)*1e6  InductivePower=load(24,3)*1e6  CapacitivePower=0  Pabc=[10e3 9e3 11e3]  QLabc=[100 90 110]  QCabc=[100 90 110]  Pabcp=[10e3 9e3 11e3]  QLabcp=[100 90 110]  QCabcp=[100 90 110]  Measurements=None  LoadType=constant PQ
  Load25 : powerlib/Elements/Three-Phase Parallel RLC Load  LConnTagsString=A|B|C  Configuration=Y (grounded)  NominalVoltage=(274783)*1.01161  Vabc=[1e3 1e3 1e3]  Vabcp=[1e3 1e3 1e3]  NominalFrequency=50  UnbalancedPower=off  ActivePower=load(25,2)*1e6  InductivePower=load(25,3)*1e6  CapacitivePower=0  Pabc=[10e3 9e3 11e3]  QLabc=[100 90 110]  QCabc=[100 90 110]  Pabcp=[10e3 9e3 11e3]  QLabcp=[100 90 110]  QCabcp=[100 90 110]  Measurements=None  LoadType=constant PQ
  Load26 : powerlib/Elements/Three-Phase Parallel RLC Load  LConnTagsString=A|B|C  Configuration=Y (grounded)  NominalVoltage=(285131)*1.0039  Vabc=[1e3 1e3 1e3]  Vabcp=[1e3 1e3 1e3]  NominalFrequency=50  UnbalancedPower=off  ActivePower=load(26,2)*1e6  InductivePower=load(26,3)*1e6  CapacitivePower=0  Pabc=[10e3 9e3 11e3]  QLabc=[100 90 110]  QCabc=[100 90 110]  Pabcp=[10e3 9e3 11e3]  QLabcp=[100 90 110]  QCabcp=[100 90 110]  Measurements=None  LoadType=constant PQ
  Load27 : powerlib/Elements/Three-Phase Parallel RLC Load  LConnTagsString=A|B|C  Configuration=Y (grounded)  NominalVoltage=(277920)*1.00693  Vabc=[1e3 1e3 1e3]  Vabcp=[1e3 1e3 1e3]  NominalFrequency=50  UnbalancedPower=off  ActivePower=load(27,2)*1e6  InductivePower=load(27,3)*1e6  CapacitivePower=0  Pabc=[10e3 9e3 11e3]  QLabc=[100 90 110]  QCabc=[100 90 110]  Pabcp=[10e3 9e3 11e3]  QLabcp=[100 90 110]  QCabcp=[100 90 110]  Measurements=None  LoadType=constant PQ
  Load28 : powerlib/Elements/Three-Phase Parallel RLC Load  LConnTagsString=A|B|C  Configuration=Y (grounded)  NominalVoltage=(276455)*1.0054  Vabc=[1e3 1e3 1e3]  Vabcp=[1e3 1e3 1e3]  NominalFrequency=50  UnbalancedPower=off  ActivePower=load(28,2)*1e6  InductivePower=load(28,3)*1e6  CapacitivePower=0  Pabc=[10e3 9e3 11e3]  QLabc=[100 90 110]  QCabc=[100 90 110]  Pabcp=[10e3 9e3 11e3]  QLabcp=[100 90 110]  QCabcp=[100 90 110]  Measurements=None  LoadType=constant PQ
  Load29 : powerlib/Elements/Three-Phase Parallel RLC Load  LConnTagsString=A|B|C  Configuration=Y (grounded)  NominalVoltage=(283244)*1.04477  Vabc=[1e3 1e3 1e3]  Vabcp=[1e3 1e3 1e3]  NominalFrequency=50  UnbalancedPower=off  ActivePower=load(29,2)*1e6  InductivePower=load(29,3)*1e6  CapacitivePower=0  Pabc=[10e3 9e3 11e3]  QLabc=[100 90 110]  QCabc=[100 90 110]  Pabcp=[10e3 9e3 11e3]  QLabcp=[100 90 110]  QCabcp=[100 90 110]  Measurements=None  LoadType=constant PQ
  Load3 : powerlib/Elements/Three-Phase Parallel RLC Load  LConnTagsString=A|B|C  Configuration=Y (grounded)  NominalVoltage=(335201)*1.00135  Vabc=[1e3 1e3 1e3]  Vabcp=[1e3 1e3 1e3]  NominalFrequency=50  UnbalancedPower=off  ActivePower=load(3,2)*1e6  InductivePower=load(3,3)*1e6  CapacitivePower=0  Pabc=[10e3 9e3 11e3]  QLabc=[100 90 110]  QCabc=[100 90 110]  Pabcp=[10e3 9e3 11e3]  QLabcp=[100 90 110]  QCabcp=[100 90 110]  Measurements=None  LoadType=constant PQ
  Load4 : powerlib/Elements/Three-Phase Parallel RLC Load  LConnTagsString=A|B|C  Configuration=Y (grounded)  NominalVoltage=(331356)*1.00056  Vabc=[1e3 1e3 1e3]  Vabcp=[1e3 1e3 1e3]  NominalFrequency=50  UnbalancedPower=off  ActivePower=load(4,2)*1e6  InductivePower=load(4,3)*1e6  CapacitivePower=0  Pabc=[10e3 9e3 11e3]  QLabc=[100 90 110]  QCabc=[100 90 110]  Pabcp=[10e3 9e3 11e3]  QLabcp=[100 90 110]  QCabcp=[100 90 110]  Measurements=None  LoadType=constant PQ
  Load5 : powerlib/Elements/Three-Phase Parallel RLC Load  LConnTagsString=A|B|C  Configuration=Y (grounded)  NominalVoltage=(332350)*1.00041  Vabc=[1e3 1e3 1e3]  Vabcp=[1e3 1e3 1e3]  NominalFrequency=50  UnbalancedPower=off  ActivePower=load(5,2)*1e6  InductivePower=load(5,3)*1e6  CapacitivePower=0  Pabc=[10e3 9e3 11e3]  QLabc=[100 90 110]  QCabc=[100 90 110]  Pabcp=[10e3 9e3 11e3]  QLabcp=[100 90 110]  QCabcp=[100 90 110]  Measurements=None  LoadType=constant PQ
  Load6 : powerlib/Elements/Three-Phase Parallel RLC Load  LConnTagsString=A|B|C  Configuration=Y (grounded)  NominalVoltage=(334046)*1.00056  Vabc=[1e3 1e3 1e3]  Vabcp=[1e3 1e3 1e3]  NominalFrequency=50  UnbalancedPower=off  ActivePower=load(6,2)*1e6  InductivePower=load(6,3)*1e6  CapacitivePower=0  Pabc=[10e3 9e3 11e3]  QLabc=[100 90 110]  QCabc=[100 90 110]  Pabcp=[10e3 9e3 11e3]  QLabcp=[100 90 110]  QCabcp=[100 90 110]  Measurements=None  LoadType=constant PQ
  Load7 : powerlib/Elements/Three-Phase Parallel RLC Load  LConnTagsString=A|B|C  Configuration=Y (grounded)  NominalVoltage=(330000)*1.02255  Vabc=[1e3 1e3 1e3]  Vabcp=[1e3 1e3 1e3]  NominalFrequency=50  UnbalancedPower=off  ActivePower=load(7,2)*1e6  InductivePower=load(7,3)*1e6  CapacitivePower=0  Pabc=[10e3 9e3 11e3]  QLabc=[100 90 110]  QCabc=[100 90 110]  Pabcp=[10e3 9e3 11e3]  QLabcp=[100 90 110]  QCabcp=[100 90 110]  Measurements=None  LoadType=constant PQ
  Load8 : powerlib/Elements/Three-Phase Parallel RLC Load  LConnTagsString=A|B|C  Configuration=Y (grounded)  NominalVoltage=(334481)*1.00032  Vabc=[1e3 1e3 1e3]  Vabcp=[1e3 1e3 1e3]  NominalFrequency=50  UnbalancedPower=off  ActivePower=load(8,2)*1e6  InductivePower=load(8,3)*1e6  CapacitivePower=0  Pabc=[10e3 9e3 11e3]  QLabc=[100 90 110]  QCabc=[100 90 110]  Pabcp=[10e3 9e3 11e3]  QLabcp=[100 90 110]  QCabcp=[100 90 110]  Measurements=None  LoadType=constant PQ
  Load9 : powerlib/Elements/Three-Phase Parallel RLC Load  LConnTagsString=A|B|C  Configuration=Y (grounded)  NominalVoltage=(330000)*1.02899  Vabc=[1e3 1e3 1e3]  Vabcp=[1e3 1e3 1e3]  NominalFrequency=50  UnbalancedPower=off  ActivePower=load(9,2)*1e6  InductivePower=load(9,3)*1e6  CapacitivePower=0  Pabc=[10e3 9e3 11e3]  QLabc=[100 90 110]  QCabc=[100 90 110]  Pabcp=[10e3 9e3 11e3]  QLabcp=[100 90 110]  QCabcp=[100 90 110]  Measurements=None  LoadType=constant PQ
  MPS_2 : Subsystem
  NPS_5 : Subsystem
  P 1-3 : Scope  NumInputPorts=2
  P 2-1 : Scope  NumInputPorts=2
  P 3-5 : Scope  NumInputPorts=2
  P 4-2 : Scope  NumInputPorts=2
  PPS_5 : Subsystem
  PSS model : Constant  Value=PSSMODEL
  SPS_4 : Subsystem
  SVC205 : factslib/Power-Electronics Based FACTS/Static Var Compensator (Phasor Type)  Seq1_Only=on  SystemNominal=[(330000)*1 50]  Pbase=100e6  Qnom="[200e6  -200e6]"  Td=4e-3  mode=Voltage regulation  Vref=1.0438  ExternalVref=off  Xs=0.01  Kp_Ki=[0 500]  Bref=-.393
      settings: SourceProductName=Simscape Power Systems  SourceProductBaseCode=PS
  SVC313 : factslib/Power-Electronics Based FACTS/Static Var Compensator (Phasor Type)  Seq1_Only=off  SystemNominal="[(220000)  50]"  Pbase=100e6  Qnom="[200e6  -200e6]"  Td=4e-3  mode=Voltage regulation  Vref=1.008  ExternalVref=off  Xs=0.01  Kp_Ki=[0 500]  Bref=0.867
      settings: SourceProductName=Simscape Power Systems  SourceProductBaseCode=PS
  "SVC412 " : factslib/Power-Electronics Based FACTS/Static Var Compensator (Phasor Type)  Seq1_Only=on  SystemNominal="[(275000)  50]"  Pbase=100e6  Qnom="[200e6  -200e6]"  Td=4e-3  mode=Voltage regulation  Vref=.9940  ExternalVref=off  Xs=0.01  Kp_Ki=[0 500]  Bref=-.522
      settings: SourceProductName=Simscape Power Systems  SourceProductBaseCode=PS
  SVC507 : factslib/Power-Electronics Based FACTS/Static Var Compensator (Phasor Type)  Seq1_Only=off  SystemNominal="[(275000)    50]"  Pbase=100e6  Qnom="[200e6  -200e6]"  Td=4e-3  mode=Voltage regulation  Vref=1.0102  ExternalVref=off  Xs=0.01  Kp_Ki=[0 250]  Bref=-.04
      settings: SourceProductName=Simscape Power Systems  SourceProductBaseCode=PS
  SVC509 : factslib/Power-Electronics Based FACTS/Static Var Compensator (Phasor Type)  Seq1_Only=off  SystemNominal="[(275000)  50]"  Pbase=100e6  Qnom="[200e6  -200e6]"  Td=4e-3  mode=Voltage regulation  Vref=1.0194  ExternalVref=off  Xs=0.01  Kp_Ki=[0 250]  Bref=-1.093
      settings: SourceProductName=Simscape Power Systems  SourceProductBaseCode=PS
  Stability Signals Yellow=G1 mag=G2 cyan=G3 red=G4 {1..10} (10 alike) : Scope
  Subsystem2 : Subsystem
  T1 : powerlib/Elements/Three-Phase Transformer (Two Windings)  Winding1Connection=Delta (D1)  Winding2Connection=Yg  CoreType=Three single-phase transformers  SetSaturation=off  Hysteresis=off  DataFile='hysteresis'  SetInitialFlux=off  Measurements=None  UNITS=pu  NominalPower=[ trans(1,6)*1e6 , 50 ]  Winding1=[ trans(1,4)*1e3, 1e-6, 0 ]  Winding2=[ trans(1,5)*1e3, 1e-6, trans(1,7) ]  Rm=500  Lm=500  L0=0.5  Saturation=[ 0,0 ; 0.0024,1.2 ; 1.0,1.52 ]  InitialFluxes=[ 0.8 , -0.8 , 0.7 ]  MoreParameters=off  BreakLoop=off  DataType=off  TransfoNumber=0
  T10 : powerlib/Elements/Three-Phase Transformer (Two Windings)  Winding1Connection=Y  Winding2Connection=Y  CoreType=Three single-phase transformers  SetSaturation=off  Hysteresis=off  DataFile='hysteresis'  SetInitialFlux=off  Measurements=None  UNITS=pu  NominalPower=[ trans(10,6)*1e6 , 50 ]  Winding1=[ trans(10,4)*1e3, 1e-6 , 0 ]  Winding2=[ trans(10,5)*1e3, 0 , trans(10,7) ]  Rm=500  Lm=500  L0=0.5  Saturation=[ 0,0 ; 0.0024,1.2 ; 1.0,1.52 ]  InitialFluxes=[ 0.8 , -0.8 , 0.7 ]  MoreParameters=off  BreakLoop=off  DataType=off  TransfoNumber=0
  T11 : powerlib/Elements/Three-Phase Transformer (Two Windings)  Winding1Connection=Y  Winding2Connection=Y  CoreType=Three single-phase transformers  SetSaturation=off  Hysteresis=off  DataFile='hysteresis'  SetInitialFlux=off  Measurements=None  UNITS=pu  NominalPower=[ trans(11,6)*1e6 , 50 ]  Winding1=[ trans(11,4)*1e3, 1e-6, 0 ]  Winding2=[ trans(11,5)*1e3, 0 , trans(11,7) ]  Rm=500  Lm=500  L0=0.5  Saturation=[ 0,0 ; 0.0024,1.2 ; 1.0,1.52 ]  InitialFluxes=[ 0.8 , -0.8 , 0.7 ]  MoreParameters=off  BreakLoop=off  DataType=off  TransfoNumber=0
  T12 : powerlib/Elements/Three-Phase Transformer (Two Windings)  Winding1Connection=Y  Winding2Connection=Y  CoreType=Three single-phase transformers  SetSaturation=off  Hysteresis=off  DataFile='hysteresis'  SetInitialFlux=off  Measurements=None  UNITS=pu  NominalPower=[ trans(12,6)*1e6 , 50 ]  Winding1=[ trans(12,4)*1e3, 1e-6, 0 ]  Winding2=[ trans(12,5)*1e3, 0 , trans(12,7)]  Rm=500  Lm=500  L0=0.5  Saturation=[ 0,0 ; 0.0024,1.2 ; 1.0,1.52 ]  InitialFluxes=[ 0.8 , -0.8 , 0.7 ]  MoreParameters=off  BreakLoop=off  DataType=off  TransfoNumber=0
  T13 : powerlib/Elements/Three-Phase Transformer (Two Windings)  Winding1Connection=Y  Winding2Connection=Y  CoreType=Three single-phase transformers  SetSaturation=off  Hysteresis=off  DataFile='hysteresis'  SetInitialFlux=off  Measurements=None  UNITS=pu  NominalPower=[ trans(13,6)*1e6 , 50 ]  Winding1=[ trans(13,4)*1e3, 1e-6, 0 ]  Winding2=[ trans(13,5)*1e3, 0 , trans(13,7) ]  Rm=500  Lm=500  L0=0.5  Saturation=[ 0,0 ; 0.0024,1.2 ; 1.0,1.52 ]  InitialFluxes=[ 0.8 , -0.8 , 0.7 ]  MoreParameters=off  BreakLoop=off  DataType=off  TransfoNumber=0
  T14 : powerlib/Elements/Three-Phase Transformer (Two Windings)  Winding1Connection=Delta (D1)  Winding2Connection=Yg  CoreType=Three single-phase transformers  SetSaturation=off  Hysteresis=off  DataFile='hysteresis'  SetInitialFlux=off  Measurements=None  UNITS=pu  NominalPower=[ trans(14,6)*1e6 , 50 ]  Winding1=[ trans(14,4)*1e3, 1e-6 , 0 ]  Winding2=[ trans(14,5)*1e3, 0 , trans(14,7) ]  Rm=500  Lm=500  L0=0.5  Saturation=[ 0,0 ; 0.0024,1.2 ; 1.0,1.52 ]  InitialFluxes=[ 0.8 , -0.8 , 0.7 ]  MoreParameters=off  BreakLoop=off  DataType=off  TransfoNumber=0
  T15 : powerlib/Elements/Three-Phase Transformer (Two Windings)  Winding1Connection=Delta (D1)  Winding2Connection=Yg  CoreType=Three single-phase transformers  SetSaturation=off  Hysteresis=off  DataFile='hysteresis'  SetInitialFlux=off  Measurements=None  UNITS=pu  NominalPower=[ trans(15,6)*1e6 , 50 ]  Winding1=[ trans(15,4)*1e3, 1e-6 , 0 ]  Winding2=[ trans(15,5)*1e3, 0 , trans(15,7) ]  Rm=500  Lm=500  L0=0.5  Saturation=[ 0,0 ; 0.0024,1.2 ; 1.0,1.52 ]  InitialFluxes=[ 0.8 , -0.8 , 0.7 ]  MoreParameters=off  BreakLoop=off  DataType=off  TransfoNumber=0
  T16 : powerlib/Elements/Three-Phase Transformer (Two Windings)  Winding1Connection=Delta (D1)  Winding2Connection=Yg  CoreType=Three single-phase transformers  SetSaturation=off  Hysteresis=off  DataFile='hysteresis'  SetInitialFlux=off  Measurements=None  UNITS=pu  NominalPower=[ trans(16,6)*1e6 , 50 ]  Winding1=[ trans(16,4)*1e3, 1e-6 , 0]  Winding2=[ trans(16,5)*1e3, 0 , trans(16,7) ]  Rm=500  Lm=500  L0=0.5  Saturation=[ 0,0 ; 0.0024,1.2 ; 1.0,1.52 ]  InitialFluxes=[ 0.8 , -0.8 , 0.7 ]  MoreParameters=off  BreakLoop=off  DataType=off  TransfoNumber=0
  T17 : powerlib/Elements/Three-Phase Transformer (Two Windings)  Winding1Connection=Delta (D1)  Winding2Connection=Yg  CoreType=Three single-phase transformers  SetSaturation=off  Hysteresis=off  DataFile='hysteresis'  SetInitialFlux=off  Measurements=None  UNITS=pu  NominalPower=[ trans(17,6)*1e6 , 50 ]  Winding1=[ trans(17,4)*1e3, 1e-6 , 0 ]  Winding2=[ trans(17,5)*1e3, 0 , trans(17,7) ]  Rm=500  Lm=500  L0=0.5  Saturation=[ 0,0 ; 0.0024,1.2 ; 1.0,1.52 ]  InitialFluxes=[ 0.8 , -0.8 , 0.7 ]  MoreParameters=off  BreakLoop=off  DataType=off  TransfoNumber=0
  T18-1 : powerlib/Elements/Three-Phase Transformer (Two Windings)  Winding1Connection=Y  Winding2Connection=Y  CoreType=Three single-phase transformers  SetSaturation=off  Hysteresis=off  DataFile='hysteresis'  SetInitialFlux=off  Measurements=None  UNITS=pu  NominalPower=[ trans(18,6)*1e6 , 50 ]  Winding1=[ trans(18,4)*1e3, 1e-6, 0 ]  Winding2=[ trans(18,5)*1e3, 0 , trans(18,7) ]  Rm=500  Lm=500  L0=0.5  Saturation=[ 0,0 ; 0.0024,1.2 ; 1.0,1.52 ]  InitialFluxes=[ 0.8 , -0.8 , 0.7 ]  MoreParameters=off  BreakLoop=off  DataType=off  TransfoNumber=0
  T18-2 : powerlib/Elements/Three-Phase Transformer (Two Windings)  Winding1Connection=Y  Winding2Connection=Y  CoreType=Three single-phase transformers  SetSaturation=off  Hysteresis=off  DataFile='hysteresis'  SetInitialFlux=off  Measurements=None  UNITS=pu  NominalPower=[ trans(18,6)*1e6 , 50 ]  Winding1=[ trans(18,4)*1e3, 1e-6, 0 ]  Winding2=[ trans(18,5)*1e3, 0 , trans(18,7) ]  Rm=500  Lm=500  L0=0.5  Saturation=[ 0,0 ; 0.0024,1.2 ; 1.0,1.52 ]  InitialFluxes=[ 0.8 , -0.8 , 0.7 ]  MoreParameters=off  BreakLoop=off  DataType=off  TransfoNumber=0
  T19 : powerlib/Elements/Three-Phase Transformer (Two Windings)  Winding1Connection=Delta (D1)  Winding2Connection=Yg  CoreType=Three single-phase transformers  SetSaturation=off  Hysteresis=off  DataFile='hysteresis'  SetInitialFlux=off  Measurements=None  UNITS=pu  NominalPower=[ trans(19,6)*1e6 , 50 ]  Winding1=[ trans(19,4)*1e3, 1e-6 , 0 ]  Winding2=[ trans(19,5)*1e3, 0 , trans(19,7) ]  Rm=500  Lm=500  L0=0.5  Saturation=[ 0,0 ; 0.0024,1.2 ; 1.0,1.52 ]  InitialFluxes=[ 0.8 , -0.8 , 0.7 ]  MoreParameters=off  BreakLoop=off  DataType=off  TransfoNumber=0
  T2 : powerlib/Elements/Three-Phase Transformer (Two Windings)  Winding1Connection=Delta (D1)  Winding2Connection=Yg  CoreType=Three single-phase transformers  SetSaturation=off  Hysteresis=off  DataFile='hysteresis'  SetInitialFlux=off  Measurements=None  UNITS=pu  NominalPower=[ trans(2,6)*1e6 , 50 ]  Winding1=[ trans(2,4)*1e3, 1e-6 , 0 ]  Winding2=[ trans(2,5)*1e3, 0 , trans(2,7) ]  Rm=500  Lm=500  L0=0.5  Saturation=[ 0,0 ; 0.0024,1.2 ; 1.0,1.52 ]  InitialFluxes=[ 0.8 , -0.8 , 0.7 ]  MoreParameters=off  BreakLoop=off  DataType=off  TransfoNumber=0
  T20 : powerlib/Elements/Three-Phase Transformer (Two Windings)  Winding1Connection=Delta (D1)  Winding2Connection=Yg  CoreType=Three single-phase transformers  SetSaturation=off  Hysteresis=off  DataFile='hysteresis'  SetInitialFlux=off  Measurements=None  UNITS=pu  NominalPower=[ trans(20,6)*1e6 , 50 ]  Winding1=[ trans(20,4)*1e3, 1e-6 , 0]  Winding2=[ trans(20,5)*1e3, 0 , trans(20,7) ]  Rm=500  Lm=500  L0=0.5  Saturation=[ 0,0 ; 0.0024,1.2 ; 1.0,1.52 ]  InitialFluxes=[ 0.8 , -0.8 , 0.7 ]  MoreParameters=off  BreakLoop=off  DataType=off  TransfoNumber=0
  T21 : powerlib/Elements/Three-Phase Transformer (Two Windings)  Winding1Connection=Delta (D1)  Winding2Connection=Yg  CoreType=Three single-phase transformers  SetSaturation=off  Hysteresis=off  DataFile='hysteresis'  SetInitialFlux=off  Measurements=None  UNITS=pu  NominalPower=[ trans(21,6)*1e6 , 50 ]  Winding1=[ trans(21,4)*1e3, 1e-6 , 0 ]  Winding2=[ trans(21,5)*1e3, 0 , trans(21,7) ]  Rm=500  Lm=500  L0=0.5  Saturation=[ 0,0 ; 0.0024,1.2 ; 1.0,1.52 ]  InitialFluxes=[ 0.8 , -0.8 , 0.7 ]  MoreParameters=off  BreakLoop=off  DataType=off  TransfoNumber=0
  T3 : powerlib/Elements/Three-Phase Transformer (Two Windings)  Winding1Connection=Delta (D1)  Winding2Connection=Yg  CoreType=Three single-phase transformers  SetSaturation=off  Hysteresis=off  DataFile='hysteresis'  SetInitialFlux=off  Measurements=None  UNITS=pu  NominalPower=[ trans(3,6)*1e6 , 50 ]  Winding1=[ trans(3,4)*1e3, 1e-6 , 0 ]  Winding2=[ trans(3,5)*1e3, 0 , trans(3,7) ]  Rm=500  Lm=500  L0=0.5  Saturation=[ 0,0 ; 0.0024,1.2 ; 1.0,1.52 ]  InitialFluxes=[ 0.8 , -0.8 , 0.7 ]  MoreParameters=off  BreakLoop=off  DataType=off  TransfoNumber=0
  T4 : powerlib/Elements/Three-Phase Transformer (Two Windings)  Winding1Connection=Delta (D1)  Winding2Connection=Yg  CoreType=Three single-phase transformers  SetSaturation=off  Hysteresis=off  DataFile='hysteresis'  SetInitialFlux=off  Measurements=None  UNITS=pu  NominalPower=[ trans(4,6)*1e6 , 50 ]  Winding1=[ trans(4,4)*1e3, 1e-6 , 0 ]  Winding2=[ trans(4,5)*1e3, 0 , trans(4,7) ]  Rm=500  Lm=500  L0=0.5  Saturation=[ 0,0 ; 0.0024,1.2 ; 1.0,1.52 ]  InitialFluxes=[ 0.8 , -0.8 , 0.7 ]  MoreParameters=off  BreakLoop=off  DataType=off  TransfoNumber=0
  T5 : powerlib/Elements/Three-Phase Transformer (Two Windings)  Winding1Connection=Delta (D1)  Winding2Connection=Yg  CoreType=Three single-phase transformers  SetSaturation=off  Hysteresis=off  DataFile='hysteresis'  SetInitialFlux=off  Measurements=None  UNITS=pu  NominalPower=[ trans(5,6)*1e6 , 50 ]  Winding1=[ trans(5,4)*1e3, 1e-6 , 0 ]  Winding2=[ trans(5,5)*1e3, 0 , trans(5,7) ]  Rm=500  Lm=500  L0=0.5  Saturation=[ 0,0 ; 0.0024,1.2 ; 1.0,1.52 ]  InitialFluxes=[ 0.8 , -0.8 , 0.7 ]  MoreParameters=off  BreakLoop=off  DataType=off  TransfoNumber=0
  T6 : powerlib/Elements/Three-Phase Transformer (Two Windings)  Winding1Connection=Y  Winding2Connection=Y  CoreType=Three single-phase transformers  SetSaturation=off  Hysteresis=off  DataFile='hysteresis'  SetInitialFlux=off  Measurements=None  UNITS=pu  NominalPower=[ trans(6,6)*1e6 , 50 ]  Winding1="[ trans(6,4)*1e3, 1e-6, 0  ]"  Winding2=[ trans(6,5)*1e3, 0 , trans(6,7)]  Rm=500  Lm=500  L0=0.5  Saturation=[ 0,0 ; 0.0024,1.2 ; 1.0,1.52 ]  InitialFluxes=[ 0.8 , -0.8 , 0.7 ]  MoreParameters=off  BreakLoop=off  DataType=off  TransfoNumber=0
  T7 : powerlib/Elements/Three-Phase Transformer (Two Windings)  Winding1Connection=Y  Winding2Connection=Y  CoreType=Three single-phase transformers  SetSaturation=off  Hysteresis=off  DataFile='hysteresis'  SetInitialFlux=off  Measurements=None  UNITS=pu  NominalPower=[ trans(7,6)*1e6 , 50 ]  Winding1=[ trans(7,4)*1e3, 1e-6, 0 ]  Winding2=[ trans(7,5)*1e3, 0 , trans(7,7) ]  Rm=500  Lm=500  L0=0.5  Saturation=[ 0,0 ; 0.0024,1.2 ; 1.0,1.52 ]  InitialFluxes=[ 0.8 , -0.8 , 0.7 ]  MoreParameters=off  BreakLoop=off  DataType=off  TransfoNumber=0
  T8 : powerlib/Elements/Three-Phase Transformer (Two Windings)  Winding1Connection=Delta (D1)  Winding2Connection=Yg  CoreType=Three single-phase transformers  SetSaturation=off  Hysteresis=off  DataFile='hysteresis'  SetInitialFlux=off  Measurements=None  UNITS=pu  NominalPower=[ trans(8,6)*1e6 , 50 ]  Winding1=[ trans(8,4)*1e3, 1e-6 , 0 ]  Winding2=[ trans(8,5)*1e3, 0 , trans(8,7)]  Rm=500  Lm=500  L0=0.5  Saturation=[ 0,0 ; 0.0024,1.2 ; 1.0,1.52 ]  InitialFluxes=[ 0.8 , -0.8 , 0.7 ]  MoreParameters=off  BreakLoop=off  DataType=off  TransfoNumber=0
  T9 : powerlib/Elements/Three-Phase Transformer (Two Windings)  Winding1Connection=Delta (D1)  Winding2Connection=Yg  CoreType=Three single-phase transformers  SetSaturation=off  Hysteresis=off  DataFile='hysteresis'  SetInitialFlux=off  Measurements=None  UNITS=pu  NominalPower=[ trans(9,6)*1e6 , 50 ]  Winding1=[ trans(9,4)*1e3, 1e-6, 0 ]  Winding2=[ trans(9,5)*1e3, 0 , trans(9,7)]  Rm=500  Lm=500  L0=0.5  Saturation=[ 0,0 ; 0.0024,1.2 ; 1.0,1.52 ]  InitialFluxes=[ 0.8 , -0.8 , 0.7 ]  MoreParameters=off  BreakLoop=off  DataType=off  TransfoNumber=0
  TPS_4 : Subsystem
  TPS_5 : Subsystem
  Three-Phase V-I Measurement{1..4} (4 alike) : powerlib/Measurements/Three-Phase V-I Measurement  VoltageMeasurement=phase-to-ground  SetLabelV=off  LabelV=Vabc  Vpu=off  VpuLL=off  CurrentMeasurement=yes  SetLabelI=off  LabelI=Iabc  Ipu=off  Pbase=100e6  Vbase=500e3  OutputType=Complex  PhasorSimulation=on  PSBequivalent=0
  VPS_2 : Subsystem
  YPS_3 : Subsystem
  powergui : powerlib/powergui  Priority=1  SimulationMode=Phasor  SampleTime=50e-6  frequency=50  Iterations=50  frequencyindice=50  Pbase=100e6  ErrMax=0.0001  UnitsV=kV  UnitsW=MW  buscounter=0  FunctionMessages=off  echomessages=off  EnableUseOfTLC=off  CurrentSourceSwitches=off  DisableSnubberDevices=off  DisableRonSwitches=off  DisableVfSwitches=off  DisplayEquations=off  SolverType=Tustin  Interpol=off  ExternalGateDelay=off  methode=off  Ts=100  x0status=blocks  SPID=off  SwTol=0  HookPort=off  RestoreLinks=warning  ResistiveCurrentMeasurement=off  Frange=[0:2:500]  Ylog=off  Xlog=on  ShowGrid=off  save=off  variable=ZData  structure=0  ZoomFFT=off  StartTime=0.0  cycles=1  DisplayStyle=1  fundamental=60  FreqAxis=off  MaxFrequency=1000  frequencyindicesteady=1  RmsSteady=1  display=off
  tag scope: PSSmodel=global
  wires:
  Demux/1 -> P 4-2/1
  Demux/2 -> P 4-2/2
  3-Phase Active & Reactive Power (Phasor Type)1/1 -> Demux/1
  Three-Phase V-I Measurement1/2 -> 3-Phase Active & Reactive Power (Phasor Type)1/2
  Three-Phase V-I Measurement1/1 -> 3-Phase Active & Reactive Power (Phasor Type)1/1
  Demux1/1 -> P 2-1/1
  Three-Phase V-I Measurement2/2 -> 3-Phase Active & Reactive Power (Phasor Type)2/2
  Three-Phase V-I Measurement2/1 -> 3-Phase Active & Reactive Power (Phasor Type)2/1
  3-Phase Active & Reactive Power (Phasor Type)2/1 -> Demux1/1
  Demux1/2 -> P 2-1/2
  Demux2/1 -> P 1-3/1
  3-Phase Active & Reactive Power (Phasor Type)3/1 -> Demux2/1
  Demux2/2 -> P 1-3/2
  Three-Phase V-I Measurement3/1 -> 3-Phase Active & Reactive Power (Phasor Type)3/1
  Three-Phase V-I Measurement3/2 -> 3-Phase Active & Reactive Power (Phasor Type)3/2
  Demux3/1 -> P 3-5/1
  3-Phase Active & Reactive Power (Phasor Type)4/1 -> Demux3/1
  Demux3/2 -> P 3-5/2
  Three-Phase V-I Measurement4/2 -> 3-Phase Active & Reactive Power (Phasor Type)4/2
  Three-Phase V-I Measurement4/1 -> 3-Phase Active & Reactive Power (Phasor Type)4/1
  PSS model/1 -> [PSSmodel]
  SVC205/1 -> Bus Selector1/1
  Bus Selector1/1 -> Stability Signals Yellow=G1 mag=G2 cyan=G3 red=G4 1/1  "<Q (pu)>"
  Bus Selector1/2 -> Stability Signals Yellow=G1 mag=G2 cyan=G3 red=G4 2/1  "<Vm (pu)>"
  "SVC412 "/1 -> Bus Selector3/1
  Bus Selector3/1 -> Stability Signals Yellow=G1 mag=G2 cyan=G3 red=G4 5/1  "<Q (pu)>"
  Bus Selector3/2 -> Stability Signals Yellow=G1 mag=G2 cyan=G3 red=G4 6/1  "<Vm (pu)>"
  SVC507/1 -> Bus Selector4/1
  Bus Selector4/1 -> Stability Signals Yellow=G1 mag=G2 cyan=G3 red=G4 7/1  "<Q (pu)>"
  Bus Selector4/2 -> Stability Signals Yellow=G1 mag=G2 cyan=G3 red=G4 8/1  "<Vm (pu)>"
  SVC509/1 -> Bus Selector5/1
  Bus Selector5/1 -> Stability Signals Yellow=G1 mag=G2 cyan=G3 red=G4 9/1  "<Q (pu)>"
  Bus Selector5/2 -> Stability Signals Yellow=G1 mag=G2 cyan=G3 red=G4 10/1  "<Vm (pu)>"
  Bus Selector2/1 -> Stability Signals Yellow=G1 mag=G2 cyan=G3 red=G4 3/1  "<Q (pu)>"
  Bus Selector2/2 -> Stability Signals Yellow=G1 mag=G2 cyan=G3 red=G4 4/1  "<Vm (pu)>"
  SVC313/1 -> Bus Selector2/1
  connections:
  L-38-1/LConn1 -- L-35-1/LConn1 -- L-35-2/LConn1 -- B406/RConn1 -- L-38-2/LConn1
  B406/RConn2 -- L-35-1/LConn2 -- L-35-2/LConn2 -- L-38-1/LConn2 -- L-38-2/LConn2
  L-35-1/LConn3 -- L-35-2/LConn3 -- B406/RConn3 -- L-38-1/LConn3 -- L-38-2/LConn3
  B407/RConn1 -- L-38-1/RConn1 -- L-38-2/RConn1
  B407/RConn2 -- L-38-1/RConn2 -- L-38-2/RConn2
  B407/RConn3 -- L-38-1/RConn3 -- L-38-2/RConn3
  B405/RConn1 -- L-35-2/RConn1 -- L-35-1/RConn1 -- T17/RConn1
  B405/RConn2 -- L-35-2/RConn2 -- L-35-1/RConn2 -- T17/RConn2
  B405/RConn3 -- L-35-2/RConn3 -- L-35-1/RConn3 -- T17/RConn3
  B407/LConn1 -- Load20/LConn1 -- L-39/LConn1 -- T16/RConn1
  B407/LConn2 -- Load20/LConn2 -- L-39/LConn2 -- T16/RConn2
  B407/LConn3 -- Load20/LConn3 -- L-39/LConn3 -- T16/RConn3
  T15/RConn1 -- B408/RConn1 -- L-39/RConn1 -- L-36-1/RConn1
  B408/RConn2 -- L-39/RConn2 -- L-36-1/RConn2 -- T15/RConn2
  B408/RConn3 -- L-39/RConn3 -- L-36-1/RConn3 -- T15/RConn3
  B405/LConn1 -- L-36-1/LConn1 -- Load18/LConn1 -- L-37-2/LConn1 -- L-37-3/LConn1 -- L-37-1/LConn1
  B405/LConn2 -- Load18/LConn2 -- L-37-2/LConn2 -- L-37-3/LConn2 -- L-36-1/LConn2 -- L-37-1/LConn2
  Load18/LConn3 -- L-37-2/LConn3 -- L-37-3/LConn3 -- L-36-1/LConn3 -- B405/LConn3 -- L-37-1/LConn3
  L-37-2/RConn1 -- L-37-1/RConn1 -- B409/RConn1 -- L-37-3/RConn1
  L-37-2/RConn2 -- L-37-1/RConn2 -- B409/RConn2 -- L-37-3/RConn2
  B409/RConn3 -- L-37-2/RConn3 -- L-37-3/RConn3 -- L-37-1/RConn3
  B409/LConn1 -- Load22/LConn1 -- Comp4-409/LConn1 -- L-41-2/LConn1 -- L-41-1/LConn1
  B409/LConn2 -- Comp4-409/LConn2 -- Load22/LConn2 -- L-41-2/LConn2 -- L-41-1/LConn2
  B409/LConn3 -- Comp4-409/LConn3 -- Load22/LConn3 -- L-41-2/LConn3 -- L-41-1/LConn3
  B408/LConn1 -- Load21/LConn1 -- L-40-2/LConn1 -- L-40-1/LConn1
  Load21/LConn2 -- L-40-2/LConn2 -- B408/LConn2 -- L-40-1/LConn2
  B408/LConn3 -- Load21/LConn3 -- L-40-2/LConn3 -- L-40-1/LConn3
  B411/RConn1 -- L-42/RConn1 -- L-41-2/RConn1 -- L-41-1/RConn1
  L-41-2/RConn2 -- L-41-1/RConn2 -- L-42/RConn2 -- B411/RConn2
  B411/RConn3 -- L-42/RConn3 -- L-41-2/RConn3 -- L-41-1/RConn3
  T14/RConn1 -- L-40-1/RConn1 -- L-40-2/RConn1 -- B410/RConn1
  B410/RConn2 -- L-40-2/RConn2 -- L-40-1/RConn2 -- T14/RConn2
  T14/RConn3 -- L-40-2/RConn3 -- L-40-1/RConn3 -- B410/RConn3
  L-44-1/LConn1 -- L-44-2/LConn1 -- L-43-1/LConn1 -- L-43-2/LConn1 -- L-43-3/LConn1 -- L-42/LConn1 -- Load23/LConn1 -- L-43-4/LConn1 -- B410/LConn1
  L-44-1/LConn2 -- L-44-2/LConn2 -- L-43-1/LConn2 -- L-43-2/LConn2 -- L-43-3/LConn2 -- L-42/LConn2 -- Load23/LConn2 -- L-43-4/LConn2 -- B410/LConn2
  L-44-1/LConn3 -- L-43-3/LConn3 -- L-42/LConn3 -- Load23/LConn3 -- L-43-4/LConn3 -- B410/LConn3 -- L-43-2/LConn3 -- L-43-1/LConn3 -- L-44-2/LConn3
  B413/RConn1 -- L-44-2/RConn1 -- L-44-1/RConn1
  B413/RConn2 -- L-44-2/RConn2 -- L-44-1/RConn2
  B413/RConn3 -- L-44-2/RConn3 -- L-44-1/RConn3
  B411/LConn1 -- Comp5-411/LConn1 -- Load24/LConn1 -- L-45-2/LConn1 -- L-45-1/LConn1
  B411/LConn2 -- Comp5-411/LConn2 -- Load24/LConn2 -- L-45-2/LConn2 -- L-45-1/LConn2
  B411/LConn3 -- Comp5-411/LConn3 -- Load24/LConn3 -- L-45-2/LConn3 -- L-45-1/LConn3
  B412/RConn1 -- L-45-2/RConn1 -- L-45-1/RConn1 -- L-43-4/RConn1 -- L-43-3/RConn1 -- L-43-1/RConn1 -- L-43-2/RConn1
  B412/RConn2 -- L-45-2/RConn2 -- L-45-1/RConn2 -- L-43-4/RConn2 -- L-43-3/RConn2 -- L-43-1/RConn2 -- L-43-2/RConn2
  L-43-3/RConn3 -- L-43-1/RConn3 -- L-43-2/RConn3 -- L-45-2/RConn3 -- L-45-1/RConn3 -- L-43-4/RConn3 -- B412/RConn3
  Load25/LConn1 -- "SVC412 "/LConn1 -- B412/LConn1
  Load25/LConn2 -- "SVC412 "/LConn2 -- B412/LConn2
  Load25/LConn3 -- "SVC412 "/LConn3 -- B412/LConn3
  B404/LConn3 -- T17/LConn3
  B404/LConn2 -- T17/LConn2
  B404/LConn1 -- T17/LConn1
  GPS_4/LConn2 -- B404/RConn2
  GPS_4/LConn1 -- B404/RConn1
  GPS_4/LConn3 -- Load Flow Bus2/LConn1 -- B404/RConn3
  B403/RConn2 -- T16/LConn2
  B403/RConn1 -- T16/LConn1
  B403/RConn3 -- T16/LConn3
  SPS_4/LConn3 -- Load Flow Bus1/LConn1 -- B403/LConn3
  SPS_4/LConn2 -- B403/LConn2
  SPS_4/LConn1 -- B403/LConn1
  CPS_4/LConn3 -- B402/LConn3
  CPS_4/LConn2 -- B402/LConn2
  B402/RConn2 -- T15/LConn2
  CPS_4/LConn1 -- Load Flow Bus3/LConn1 -- B402/LConn1
  B402/RConn3 -- T15/LConn3
  B402/RConn1 -- T15/LConn1
  B401/RConn2 -- T14/LConn2
  B401/RConn3 -- T14/LConn3
  B401/RConn1 -- T14/LConn1
  TPS_4/LConn1 -- Load Flow Bus4/LConn1 -- B401/LConn1
  TPS_4/LConn2 -- B401/LConn2
  TPS_4/LConn3 -- B401/LConn3
  B413/LConn1 -- T18-2/LConn1 -- T18-1/LConn1
  B413/LConn2 -- T18-2/LConn2 -- T18-1/LConn2
  B413/LConn3 -- T18-2/LConn3 -- T18-1/LConn3
  B414/RConn2 -- T18-2/RConn2 -- T18-1/RConn2
  B414/RConn1 -- T18-2/RConn1 -- T18-1/RConn1
  B414/RConn3 -- T18-2/RConn3 -- T18-1/RConn3
  B415/RConn1 -- L-46-2/RConn1 -- L-46-1/RConn1
  B415/RConn2 -- L-46-2/RConn2 -- L-46-1/RConn2
  B415/RConn3 -- L-46-2/RConn3 -- L-46-1/RConn3
  B414/LConn1 -- Comp6-414/LConn1 -- L-46-2/LConn1 -- L-46-1/LConn1
  Comp6-414/LConn2 -- B414/LConn2 -- L-46-1/LConn2 -- L-46-2/LConn2
  B414/LConn3 -- Comp6-414/LConn3 -- L-46-2/LConn3 -- L-46-1/LConn3
  L-6-1/RConn1 -- Three-Phase V-I Measurement1/LConn1 -- L-6-2/RConn1
  L-6-1/RConn2 -- L-6-2/RConn2 -- Three-Phase V-I Measurement1/LConn2
  L-6-1/RConn3 -- L-6-2/RConn3 -- Three-Phase V-I Measurement1/LConn3
  B416/LConn1 -- Comp8-416/LConn1 -- L-6-2/LConn1 -- L-6-1/LConn1
  B416/LConn2 -- Comp8-416/LConn2 -- L-6-2/LConn2 -- L-6-1/LConn2
  B416/LConn3 -- Comp8-416/LConn3 -- L-6-2/LConn3 -- L-6-1/LConn3
  L-7-1/RConn1 -- B206/RConn1 -- L-5-1/RConn1 -- L-5-2/RConn1 -- T2/RConn1 -- L-7-2/RConn1
  B206/RConn2 -- L-5-2/RConn2 -- L-5-1/RConn2 -- L-7-1/RConn2 -- L-7-2/RConn2 -- T2/RConn2
  T2/RConn3 -- L-7-1/RConn3 -- L-7-2/RConn3 -- L-5-2/RConn3 -- L-5-1/RConn3 -- B206/RConn3
  Load2/LConn1 -- L-5-1/LConn1 -- SVC205/LConn1 -- B205/LConn1 -- L-5-2/LConn1
  Load2/LConn2 -- L-5-1/LConn2 -- SVC205/LConn2 -- B205/LConn2 -- L-5-2/LConn2
  Load2/LConn3 -- L-5-1/LConn3 -- SVC205/LConn3 -- L-5-2/LConn3 -- B205/LConn3
  BPS_2/LConn1 -- B201/RConn1
  B201/LConn1 -- T2/LConn1
  BPS_2/LConn3 -- Load Flow Bus6/LConn1 -- B201/RConn3
  B201/LConn2 -- T2/LConn2
  B201/LConn3 -- T2/LConn3
  BPS_2/LConn2 -- B201/RConn2
  B207/LConn1 -- L-11/LConn1 -- L-7-2/LConn1 -- L-7-1/LConn1
  B207/LConn2 -- L-11/LConn2 -- L-7-2/LConn2 -- L-7-1/LConn2
  B207/LConn3 -- L-11/LConn3 -- L-7-2/LConn3 -- L-7-1/LConn3
  B207/RConn1 -- L-10-2/RConn1 -- L-10-1/RConn1 -- Load4/LConn1
  B207/RConn2 -- L-10-2/RConn2 -- L-10-1/RConn2 -- Load4/LConn2
  B207/RConn3 -- L-10-2/RConn3 -- L-10-1/RConn3 -- Load4/LConn3
  T4/RConn1 -- L-10-1/LConn1 -- L-10-2/LConn1 -- B208/RConn1
  T4/RConn2 -- L-10-1/LConn2 -- L-10-2/LConn2 -- B208/RConn2
  T4/RConn3 -- L-10-1/LConn3 -- L-10-2/LConn3 -- B208/RConn3
  VPS_2/LConn1 -- B203/RConn1
  B203/LConn1 -- T4/LConn1
  B203/LConn3 -- T4/LConn3
  VPS_2/LConn2 -- B203/RConn2
  VPS_2/LConn3 -- Load Flow Bus5/LConn1 -- B203/RConn3
  B203/LConn2 -- T4/LConn2
  L-12-3/LConn1 -- L-12-2/LConn1 -- L-12-1/LConn1 -- B211/RConn1
  L-12-3/LConn2 -- L-12-2/LConn2 -- L-12-1/LConn2 -- B211/RConn2
  L-12-3/LConn3 -- L-12-2/LConn3 -- B211/RConn3 -- L-12-1/LConn3
  Load5/LConn1 -- L-12-3/RConn1 -- L-12-2/RConn1 -- L-12-1/RConn1 -- B208/LConn1
  Load5/LConn2 -- L-12-3/RConn2 -- L-12-1/RConn2 -- B208/LConn2 -- L-12-2/RConn2
  Load5/LConn3 -- L-12-3/RConn3 -- L-12-2/RConn3 -- L-12-1/RConn3 -- B208/LConn3
  B211/LConn1 -- Load6/LConn1 -- L-16/RConn1 -- L-15-2/RConn1 -- L-15-1/RConn1
  L-16/RConn2 -- Load6/LConn2 -- L-15-2/RConn2 -- L-15-1/RConn2 -- B211/LConn2
  B211/LConn3 -- Load6/LConn3 -- L-16/RConn3 -- L-15-2/RConn3 -- L-15-1/RConn3
  B206/LConn1 -- L-9-1/RConn1 -- L-9-2/RConn1 -- Load3/LConn1 -- L-8-2/RConn1 -- L-8-1/RConn1
  L-9-1/RConn2 -- Load3/LConn2 -- L-8-2/RConn2 -- L-8-1/RConn2 -- B206/LConn2 -- L-9-2/RConn2
  B206/LConn3 -- L-9-1/RConn3 -- L-9-2/RConn3 -- Load3/LConn3 -- L-8-2/RConn3 -- L-8-1/RConn3
  L-15-2/LConn1 -- L-15-1/LConn1 -- L-8-1/LConn1 -- L-13/LConn1 -- B212/RConn1 -- L-8-2/LConn1
  B212/RConn2 -- L-13/LConn2 -- L-8-2/LConn2 -- L-15-2/LConn2 -- L-15-1/LConn2 -- L-8-1/LConn2
  L-15-2/LConn3 -- L-15-1/LConn3 -- L-8-2/LConn3 -- L-8-1/LConn3 -- L-13/LConn3 -- B212/RConn3
  T3/RConn3 -- L-11/RConn3 -- B209/RConn3
  T3/RConn2 -- L-11/RConn2 -- B209/RConn2
  T3/RConn1 -- L-11/RConn1 -- B209/RConn1
  B202/LConn2 -- T3/LConn2
  EPS_2/LConn3 -- B202/RConn3
  B202/LConn3 -- T3/LConn3
  EPS_2/LConn1 -- Load Flow Bus7/LConn1 -- B202/RConn1
  B202/LConn1 -- T3/LConn1
  EPS_2/LConn2 -- B202/RConn2
  T6/LConn1 -- L-13/RConn1 -- B209/LConn1
  T6/LConn2 -- L-13/RConn2 -- B209/LConn2
  T6/LConn3 -- L-13/RConn3 -- B209/LConn3
  B210/RConn1 -- T6/RConn1
  B210/RConn2 -- T6/RConn2
  B210/RConn3 -- T6/RConn3
  B213/RConn1 -- L-14-1/LConn1 -- L-14-2/LConn1
  B213/RConn2 -- L-14-1/LConn2 -- L-14-2/LConn2
  B213/RConn3 -- L-14-1/LConn3 -- L-14-2/LConn3
  B210/LConn1 -- L-14-2/RConn1 -- L-14-1/RConn1
  B210/LConn2 -- L-14-2/RConn2 -- L-14-1/RConn2
  B210/LConn3 -- L-14-2/RConn3 -- L-14-1/RConn3
  L-17/RConn1 -- Comp2-212/LConn1 -- Load7/LConn1 -- B212/LConn1
  B212/LConn2 -- Load7/LConn2 -- Comp2-212/LConn2 -- L-17/RConn2
  B212/LConn3 -- Load7/LConn3 -- Comp2-212/LConn3 -- L-17/RConn3
  B214/RConn2 -- L-16/LConn2 -- T7/RConn2
  B214/RConn1 -- L-16/LConn1 -- T7/RConn1
  B214/RConn3 -- L-16/LConn3 -- T7/RConn3
  T7/LConn1 -- B213/LConn1
  T7/LConn2 -- B213/LConn2
  T7/LConn3 -- B213/LConn3
  L-18/LConn2 -- L-20-1/LConn2 -- L-20-2/LConn2 -- B216/RConn2
  L-18/LConn1 -- L-20-1/LConn1 -- L-20-2/LConn1 -- B216/RConn1
  L-18/LConn3 -- B216/RConn3 -- L-20-1/LConn3 -- L-20-2/LConn3
  B214/LConn3 -- L-19/RConn3 -- L-18/RConn3
  B214/LConn1 -- L-19/RConn1 -- L-18/RConn1
  B214/LConn2 -- L-19/RConn2 -- L-18/RConn2
  L-22/LConn1 -- L-19/LConn1 -- L-17/LConn1 -- L-21-2/LConn1 -- L-21-1/LConn1 -- B217/RConn1
  L-22/LConn2 -- L-19/LConn2 -- L-17/LConn2 -- L-21-1/LConn2 -- L-21-2/LConn2 -- B217/RConn2
  L-22/LConn3 -- L-19/LConn3 -- L-17/LConn3 -- L-21-1/LConn3 -- L-21-2/LConn3 -- B217/RConn3
  L-22/RConn1 -- Comp3-216/LConn1 -- Load9/LConn1 -- B216/LConn1
  L-22/RConn2 -- Comp3-216/LConn2 -- Load9/LConn2 -- B216/LConn2
  L-22/RConn3 -- Comp3-216/LConn3 -- Load9/LConn3 -- B216/LConn3
  B215/RConn1 -- L-9-2/LConn1 -- L-9-1/LConn1
  B215/RConn2 -- L-9-2/LConn2 -- L-9-1/LConn2
  B215/RConn3 -- L-9-2/LConn3 -- L-9-1/LConn3
  T5/RConn1 -- Load8/LConn1 -- L-20-2/RConn1 -- L-20-1/RConn1 -- L-21-1/RConn1 -- L-21-2/RConn1 -- B215/LConn1
  T5/RConn2 -- Load8/LConn2 -- L-20-2/RConn2 -- L-20-1/RConn2 -- L-21-1/RConn2 -- L-21-2/RConn2 -- B215/LConn2
  T5/RConn3 -- Load8/LConn3 -- L-20-2/RConn3 -- L-20-1/RConn3 -- L-21-1/RConn3 -- L-21-2/RConn3 -- B215/LConn3
  L-2-1/RConn1 -- L-1-1/RConn1 -- L-1-2/RConn1 -- L-2-2/RConn1 -- Three-Phase V-I Measurement2/LConn1
  L-2-2/RConn3 -- Three-Phase V-I Measurement2/LConn3 -- L-1-1/RConn3 -- L-1-2/RConn3 -- L-2-1/RConn3
  L-1-1/LConn1 -- B217/LConn1 -- Load10/LConn1 -- L-2-2/LConn1 -- L-2-1/LConn1 -- L-1-2/LConn1
  B217/LConn2 -- Load10/LConn2 -- L-2-2/LConn2 -- L-2-1/LConn2 -- L-1-2/LConn2 -- L-1-1/LConn2
  L-1-1/LConn3 -- Load10/LConn3 -- L-2-2/LConn3 -- L-2-1/LConn3 -- L-1-2/LConn3 -- B217/LConn3
  L-3-1/RConn1 -- L-4/RConn1 -- L-3-2/RConn1 -- Three-Phase V-I Measurement3/LConn1
  L-3-1/RConn2 -- L-4/RConn2 -- L-3-2/RConn2 -- Three-Phase V-I Measurement3/LConn2
  L-3-1/RConn3 -- L-4/RConn3 -- L-3-2/RConn3 -- Three-Phase V-I Measurement3/LConn3
  B102/LConn1 -- L-3-1/LConn1 -- T1/RConn1 -- Load1/LConn1 -- L-4/LConn1 -- L-3-2/LConn1
  B102/LConn2 -- L-3-1/LConn2 -- T1/RConn2 -- Load1/LConn2 -- L-4/LConn2 -- L-3-2/LConn2
  B102/LConn3 -- L-3-1/LConn3 -- T1/RConn3 -- Load1/LConn3 -- L-4/LConn3 -- L-3-2/LConn3
  HPS_1/LConn1 -- B101/RConn1
  B101/LConn1 -- T1/LConn1
  HPS_1/LConn3 -- Load Flow Bus9/LConn1 -- B101/RConn3
  HPS_1/LConn2 -- B101/RConn2
  B101/LConn3 -- T1/LConn3
  B101/LConn2 -- T1/LConn2
  L-30-2/LConn2 -- B309/LConn2 -- Load14/LConn2 -- L-30-1/LConn2
  L-30-2/LConn3 -- B309/LConn3 -- Load14/LConn3 -- L-30-1/LConn3
  T11/LConn1 -- T12/LConn1 -- B305/RConn1 -- L-24-1/LConn1 -- L-24-2/LConn1 -- L-25/LConn1
  T11/LConn2 -- T12/LConn2 -- B305/RConn2 -- L-24-1/LConn2 -- L-24-2/LConn2 -- L-25/LConn2
  T11/LConn3 -- T12/LConn3 -- B305/RConn3 -- L-24-1/LConn3 -- L-24-2/LConn3 -- L-25/LConn3
  L-24-2/RConn1 -- L-24-1/RConn1 -- L-23/RConn1 -- B303/RConn1
  L-24-2/RConn2 -- L-24-1/RConn2 -- L-23/RConn2 -- B303/RConn2
  L-24-2/RConn3 -- L-24-1/RConn3 -- L-23/RConn3 -- B303/RConn3
  B307/RConn1 -- L-28/LConn1 -- L-27-2/LConn1 -- L-27-1/LConn1
  B307/RConn2 -- L-28/LConn2 -- L-27-2/LConn2 -- L-27-1/LConn2
  B307/RConn3 -- L-28/LConn3 -- L-27-2/LConn3 -- L-27-1/LConn3
  B305/LConn1 -- L-26/RConn1 -- L-27-2/RConn1 -- L-27-1/RConn1
  B305/LConn2 -- L-26/RConn2 -- L-27-2/RConn2 -- L-27-1/RConn2
  B305/LConn3 -- L-26/RConn3 -- L-27-2/RConn3 -- L-27-1/RConn3
  L-25/RConn1 -- B304/LConn1
  L-25/RConn2 -- B304/LConn2
  L-25/RConn3 -- B304/LConn3
  LPS_3/LConn2 -- B301/LConn2
  LPS_3/LConn1 -- B301/LConn1
  LPS_3/LConn3 -- Load Flow Bus10/LConn1 -- B301/LConn3
  T8/LConn1 -- B301/RConn1
  T8/LConn3 -- B301/RConn3
  T8/LConn2 -- B301/RConn2
  T8/RConn1 -- B303/LConn1
  T8/RConn2 -- B303/LConn2
  T8/RConn3 -- B303/LConn3
  B304/RConn1 -- L-23/LConn1 -- T10/LConn1
  B304/RConn2 -- L-23/LConn2 -- T10/LConn2
  T10/LConn3 -- L-23/LConn3 -- B304/RConn3
  L-33/LConn1 -- B314/RConn1
  L-33/LConn2 -- B314/RConn2
  L-33/LConn3 -- B314/RConn3
  L-33/RConn1 -- SVC313/LConn1 -- B313/LConn1
  L-33/RConn2 -- SVC313/LConn2 -- B313/LConn2
  L-33/RConn3 -- SVC313/LConn3 -- B313/LConn3
  T12/RConn3 -- Load17/LConn3 -- B314/LConn3
  T12/RConn2 -- Load17/LConn2 -- B314/LConn2
  T12/RConn1 -- Load17/LConn1 -- B314/LConn1
  T10/RConn1 -- B313/RConn1 -- Load16/LConn1 -- L-32/LConn1
  B313/RConn2 -- Load16/LConn2 -- L-32/LConn2 -- T10/RConn2
  T10/RConn3 -- B313/RConn3 -- Load16/LConn3 -- L-32/LConn3
  B312/LConn2 -- Load15/LConn2 -- L-32/RConn2
  L-32/RConn1 -- B312/LConn1 -- Load15/LConn1
  L-32/RConn3 -- B312/LConn3 -- Load15/LConn3
  YPS_3/LConn3 -- B302/LConn3 -- Load Flow Bus11/LConn1
  T9/LConn3 -- B302/RConn3
  B312/RConn3 -- T9/RConn3
  T9/LConn2 -- B302/RConn2
  T9/LConn1 -- B302/RConn1
  B312/RConn2 -- T9/RConn2
  YPS_3/LConn1 -- B302/LConn1
  YPS_3/LConn2 -- B302/LConn2
  B312/RConn1 -- T9/RConn1
  B306/RConn1 -- L-26/LConn1 -- Load11/LConn1
  L-26/LConn2 -- Load11/LConn2 -- B306/RConn2
  B306/RConn3 -- L-26/LConn3 -- Load11/LConn3
  L-28/RConn1 -- B306/LConn1
  L-28/RConn2 -- B306/LConn2
  L-28/RConn3 -- B306/LConn3
  T11/RConn1 -- B311/LConn1
  T11/RConn2 -- B311/LConn2
  T11/RConn3 -- B311/LConn3
  B308/LConn1 -- Load13/LConn1 -- T13/LConn1
  B308/LConn2 -- Load13/LConn2 -- T13/LConn2
  B308/LConn3 -- Load13/LConn3 -- T13/LConn3
  T13/RConn1 -- B315/LConn1
  T13/RConn2 -- B315/LConn2
  T13/RConn3 -- B315/LConn3
  L-49-2/LConn1 -- B504/LConn1 -- L-48-1/LConn1 -- L-48-2/LConn1 -- L-49-1/LConn1
  L-49-2/LConn2 -- L-49-1/LConn2 -- L-48-1/LConn2 -- B504/LConn2 -- L-48-2/LConn2
  L-49-2/LConn3 -- L-49-1/LConn3 -- B504/LConn3 -- L-48-1/LConn3 -- L-48-2/LConn3
  B507/RConn2 -- SVC507/LConn2 -- Load27/LConn2 -- L-50-1/LConn2 -- L-48-2/RConn2 -- L-48-1/RConn2
  B507/RConn1 -- SVC507/LConn1 -- Load27/LConn1 -- L-48-2/RConn1 -- L-48-1/RConn1 -- L-50-1/LConn1
  B507/RConn3 -- SVC507/LConn3 -- Load27/LConn3 -- L-48-2/RConn3 -- L-48-1/RConn3 -- L-50-1/LConn3
  B509/RConn1 -- L-55-2/RConn1 -- L-55-1/RConn1
  B509/RConn2 -- L-55-2/RConn2 -- L-55-1/RConn2
  B509/RConn3 -- L-55-2/RConn3 -- L-55-1/RConn3
  L-55-2/LConn1 -- L-54/LConn1 -- L-55-1/LConn1 -- L-52/LConn1 -- B507/LConn1
  B507/LConn2 -- L-55-1/LConn2 -- L-52/LConn2 -- L-54/LConn2 -- L-55-2/LConn2
  L-54/LConn3 -- L-55-2/LConn3 -- B507/LConn3 -- L-55-1/LConn3 -- L-52/LConn3
  L-34-1/RConn1 -- L-34-2/RConn1 -- Three-Phase V-I Measurement4/RConn1
  L-34-1/RConn2 -- L-34-2/RConn2 -- Three-Phase V-I Measurement4/RConn2
  L-34-1/RConn3 -- L-34-2/RConn3 -- Three-Phase V-I Measurement4/RConn3
  B509/LConn1 -- Load29/LConn1 -- SVC509/LConn1 -- L-34-1/LConn1 -- L-34-2/LConn1
  Load29/LConn2 -- SVC509/LConn2 -- L-34-2/LConn2 -- L-34-1/LConn2 -- B509/LConn2
  B509/LConn3 -- L-34-1/LConn3 -- SVC509/LConn3 -- Load29/LConn3 -- L-34-2/LConn3
  PPS_5/LConn3 -- Load Flow Bus12/LConn1 -- B503/LConn3
  PPS_5/LConn1 -- B503/LConn1
  B503/RConn2 -- T21/LConn2
  B503/RConn3 -- T21/LConn3
  B503/RConn1 -- T21/LConn1
  PPS_5/LConn2 -- B503/LConn2
  B506/RConn1 -- L-53/RConn1 -- L-52/RConn1
  B506/RConn2 -- L-53/RConn2 -- L-52/RConn2
  B506/RConn3 -- L-53/RConn3 -- L-52/RConn3
  B506/LConn2 -- T21/RConn2
  B506/LConn3 -- T21/RConn3
  B506/LConn1 -- T21/RConn1
  L-49-2/RConn1 -- L-49-1/RConn1 -- L-51/RConn1 -- L-54/RConn1 -- L-53/LConn1 -- B508/RConn1
  L-49-2/RConn2 -- L-49-1/RConn2 -- L-51/RConn2 -- L-54/RConn2 -- L-53/LConn2 -- B508/RConn2
  L-49-2/RConn3 -- L-49-1/RConn3 -- L-51/RConn3 -- L-54/RConn3 -- L-53/LConn3 -- B508/RConn3
  Load28/LConn1 -- B508/LConn1
  Load28/LConn2 -- B508/LConn2
  Load28/LConn3 -- B508/LConn3
  B505/RConn1 -- L-51/LConn1 -- L-50-1/RConn1
  B505/RConn2 -- L-51/LConn2 -- L-50-1/RConn2
  B505/RConn3 -- L-51/LConn3 -- L-50-1/RConn3
  B505/LConn3 -- T20/RConn3
  B502/RConn2 -- T20/LConn2
  B502/RConn1 -- T20/LConn1
  TPS_5/LConn1 -- B502/LConn1
  TPS_5/LConn3 -- Load Flow Bus13/LConn1 -- B502/LConn3
  TPS_5/LConn2 -- B502/LConn2
  B505/LConn2 -- T20/RConn2
  B502/RConn3 -- T20/LConn3
  B505/LConn1 -- T20/RConn1
  NPS_5/LConn1 -- B501/RConn1
  B501/LConn2 -- T19/LConn2
  B501/LConn3 -- T19/LConn3
  NPS_5/LConn3 -- Load Flow Bus14/LConn1 -- B501/RConn3
  NPS_5/LConn2 -- B501/RConn2
  B501/LConn1 -- T19/LConn1
  B504/RConn2 -- Load26/LConn2 -- T19/RConn2
  B504/RConn1 -- Load26/LConn1 -- T19/RConn1
  B504/RConn3 -- Load26/LConn3 -- T19/RConn3
  Load19/LConn1 -- B406/LConn1
  Load19/LConn2 -- B406/LConn2
  Load19/LConn3 -- B406/LConn3
  B204/LConn3 -- T5/LConn3
  MPS_2/LConn1 -- Load Flow Bus8/LConn1 -- B204/RConn1
  MPS_2/LConn3 -- B204/RConn3
  MPS_2/LConn2 -- B204/RConn2
  B204/LConn1 -- T5/LConn1
  B204/LConn2 -- T5/LConn2
  B415/LConn1 -- Comp7-415/LConn1 -- L-47-2/LConn1 -- L-47-1/LConn1
  B415/LConn2 -- Comp7-415/LConn2 -- L-47-2/LConn2 -- L-47-1/LConn2
  B415/LConn3 -- Comp7-415/LConn3 -- L-47-2/LConn3 -- L-47-1/LConn3
  B416/RConn2 -- L-47-1/RConn2 -- L-47-2/RConn2
  B416/RConn3 -- L-47-1/RConn3 -- L-47-2/RConn3
  B416/RConn1 -- L-47-1/RConn1 -- L-47-2/RConn1
  B308/RConn1 -- L-29-1/LConn1 -- L-29-2/LConn1
  B308/RConn2 -- L-29-1/LConn2 -- L-29-2/LConn2
  B308/RConn3 -- L-29-1/LConn3 -- L-29-2/LConn3
  B307/LConn1 -- Load12/LConn1 -- L-29-1/RConn1 -- L-29-2/RConn1
  B307/LConn2 -- Load12/LConn2 -- L-29-1/RConn2 -- L-29-2/RConn2
  B307/LConn3 -- Load12/LConn3 -- L-29-1/RConn3 -- L-29-2/RConn3
  B205/RConn3 -- Three-Phase V-I Measurement1/RConn3
  B205/RConn2 -- Three-Phase V-I Measurement1/RConn2
  B205/RConn1 -- Three-Phase V-I Measurement1/RConn1
  L-30-2/LConn1 -- L-30-1/LConn1 -- B309/LConn1 -- Load14/LConn1
  2/RConn1 -- B310/LConn1 -- 1/RConn1
  1/RConn2 -- 2/RConn2 -- B310/LConn2
  2/RConn3 -- B310/LConn3 -- 1/RConn3
  2/LConn1 -- B311/RConn1 -- 1/LConn1
  2/LConn2 -- B311/RConn2 -- 1/LConn2
  1/LConn3 -- 2/LConn3 -- B311/RConn3
  L-2-1/RConn2 -- L-1-1/RConn2 -- L-1-2/RConn2 -- Three-Phase V-I Measurement2/LConn2 -- L-2-2/RConn2
  B102/RConn1 -- Three-Phase V-I Measurement2/RConn1
  B102/RConn2 -- Three-Phase V-I Measurement2/RConn2
  B102/RConn3 -- Three-Phase V-I Measurement2/RConn3
  L-30-1/RConn1 -- L-30-2/RConn1 -- B310/RConn1
  L-30-1/RConn2 -- L-30-2/RConn2 -- B310/RConn2
  L-30-1/RConn3 -- L-30-2/RConn3 -- B310/RConn3
  Three-Phase V-I Measurement3/RConn1 -- B309/RConn1
  Three-Phase V-I Measurement3/RConn2 -- B309/RConn2
  Three-Phase V-I Measurement3/RConn3 -- B309/RConn3
  B315/RConn3 -- Three-Phase V-I Measurement4/LConn3
  B315/RConn2 -- Three-Phase V-I Measurement4/LConn2
  B315/RConn1 -- Three-Phase V-I Measurement4/LConn1
